simulink library "AEMS_Standard_Library"  (R2016b)
(part 13 of 39)

      | bit_ext_b7 = find_system(lib_path,'LookUnderMasks','all','FollowLinks','on','Name','DEM_LIB_BIT_EXTRACT7');
      | bit_ext_b8 = find_system(lib_path,'LookUnderMasks','all','FollowLinks','on','Name','DEM_LIB_BIT_EXTRACT8');
      | bit_ext_b0 = find_system(lib_path,'LookUnderMasks','all','FollowLinks','on','Name','DEM_LIB_BIT_EXTRACT0');
      | 
      | switch LibType
      |     case '_DGN'
      |         if ismember(get_param(bit_ext_b1,'MaskType'),{'AEMS_DEM_LIB_BIT_EXTRACT'})
      |         else
      |             replace_block(lib_path,'FollowLinks','on','Name','DEM_LIB_BIT_EXTRACT1','library/SUB/DEM_LIB_BIT_EXTRACT','noprompt');
      |             replace_block(lib_path,'FollowLinks','on','Name','DEM_LIB_BIT_EXTRACT2','library/SUB/DEM_LIB_BIT_EXTRACT','noprompt');
      |             replace_block(lib_path,'FollowLinks','on','Name','DEM_LIB_BIT_EXTRACT3','library/SUB/DEM_LIB_BIT_EXTRACT','noprompt');
      |             replace_block(lib_path,'FollowLinks','on','Name','DEM_LIB_BIT_EXTRACT4','library/SUB/DEM_LIB_BIT_EXTRACT','noprompt');
      |             replace_block(lib_path,'FollowLinks','on','Name','DEM_LIB_BIT_EXTRACT5','library/SUB/DEM_LIB_BIT_EXTRACT','noprompt');
      |             replace_block(lib_path,'FollowLinks','on','Name','DEM_LIB_BIT_EXTRACT6','library/SUB/DEM_LIB_BIT_EXTRACT','noprompt');
      |             replace_block(lib_path,'FollowLinks','on','Name','DEM_LIB_BIT_EXTRACT7','library/SUB/DEM_LIB_BIT_EXTRACT','noprompt');
      |             replace_block(lib_path,'FollowLinks','on','Name','DEM_LIB_BIT_EXTRACT8','library/SUB/DEM_LIB_BIT_EXTRACT','noprompt');
      |             replace_block(lib_path,'FollowLinks','on','Name','DEM_LIB_BIT_EXTRACT0','library/SUB/DEM_LIB_BIT_EXTRACT','noprompt');
      |         end
      |         set_param([bit_ext_b1{:}],'extract_bit','132');
      |         set_param([bit_ext_b2{:}],'extract_bit','132');
      |         set_param([bit_ext_b3{:}],'extract_bit','132');
      |         set_param([bit_ext_b4{:}],'extract_bit','132');
      |         set_param([bit_ext_b5{:}],'extract_bit','132');
      |         set_param([bit_ext_b6{:}],'extract_bit','132');
      |         set_param([bit_ext_b7{:}],'extract_bit','132');
      |         set_param([bit_ext_b8{:}],'extract_bit','132');
      |         set_param([bit_ext_b0{:}],'extract_bit','132');
      |     case '_FS(Hold at Key On)'
      |         if ismember(get_param(bit_ext_b1,'MaskType'),{'AEMS_DEM_LIB_BIT_EXTRACT'})
      |         else
      |             replace_block(lib_path,'FollowLinks','on','Name','DEM_LIB_BIT_EXTRACT1','library/SUB/DEM_LIB_BIT_EXTRACT','noprompt');
      |             replace_block(lib_path,'FollowLinks','on','Name','DEM_LIB_BIT_EXTRACT2','library/SUB/DEM_LIB_BIT_EXTRACT','noprompt');
      |             replace_block(lib_path,'FollowLinks','on','Name','DEM_LIB_BIT_EXTRACT3','library/SUB/DEM_LIB_BIT_EXTRACT','noprompt');
      |             replace_block(lib_path,'FollowLinks','on','Name','DEM_LIB_BIT_EXTRACT4','library/SUB/DEM_LIB_BIT_EXTRACT','noprompt');
      |             replace_block(lib_path,'FollowLinks','on','Name','DEM_LIB_BIT_EXTRACT5','library/SUB/DEM_LIB_BIT_EXTRACT','noprompt');
      |             replace_block(lib_path,'FollowLinks','on','Name','DEM_LIB_BIT_EXTRACT6','library/SUB/DEM_LIB_BIT_EXTRACT','noprompt');
      |             replace_block(lib_path,'FollowLinks','on','Name','DEM_LIB_BIT_EXTRACT7','library/SUB/DEM_LIB_BIT_EXTRACT','noprompt');
      |             replace_block(lib_path,'FollowLinks','on','Name','DEM_LIB_BIT_EXTRACT8','library/SUB/DEM_LIB_BIT_EXTRACT','noprompt');
      |             replace_block(lib_path,'FollowLinks','on','Name','DEM_LIB_BIT_EXTRACT0','library/SUB/DEM_LIB_BIT_EXTRACT','noprompt');
      |         end
      |         set_param([bit_ext_b1{:}],'extract_bit','1');
      |         set_param([bit_ext_b2{:}],'extract_bit','1');
      |         set_param([bit_ext_b3{:}],'extract_bit','1');
      |         set_param([bit_ext_b4{:}],'extract_bit','1');
      |         set_param([bit_ext_b5{:}],'extract_bit','1');
      |         set_param([bit_ext_b6{:}],'extract_bit','1');
      |         set_param([bit_ext_b7{:}],'extract_bit','1');
      |         set_param([bit_ext_b8{:}],'extract_bit','1');
      |         set_param([bit_ext_b0{:}],'extract_bit','1');
      |     case '_FS(Reset at Key On)'
      |         if ismember(get_param(bit_ext_b1,'MaskType'),{'AEMS_DEM_LIB_BIT_EXTRACT_FS_RESET'})
      |         else
      |             replace_block(lib_path,'FollowLinks','on','Name','DEM_LIB_BIT_EXTRACT1','library/SUB/DEM_LIB_BIT_EXTRACT_FS_RESET','noprompt');
      |             replace_block(lib_path,'FollowLinks','on','Name','DEM_LIB_BIT_EXTRACT2','library/SUB/DEM_LIB_BIT_EXTRACT_FS_RESET','noprompt');
      |             replace_block(lib_path,'FollowLinks','on','Name','DEM_LIB_BIT_EXTRACT3','library/SUB/DEM_LIB_BIT_EXTRACT_FS_RESET','noprompt');
      |             replace_block(lib_path,'FollowLinks','on','Name','DEM_LIB_BIT_EXTRACT4','library/SUB/DEM_LIB_BIT_EXTRACT_FS_RESET','noprompt');
      |             replace_block(lib_path,'FollowLinks','on','Name','DEM_LIB_BIT_EXTRACT5','library/SUB/DEM_LIB_BIT_EXTRACT_FS_RESET','noprompt');
      |             replace_block(lib_path,'FollowLinks','on','Name','DEM_LIB_BIT_EXTRACT6','library/SUB/DEM_LIB_BIT_EXTRACT_FS_RESET','noprompt');
      |             replace_block(lib_path,'FollowLinks','on','Name','DEM_LIB_BIT_EXTRACT7','library/SUB/DEM_LIB_BIT_EXTRACT_FS_RESET','noprompt');
      |             replace_block(lib_path,'FollowLinks','on','Name','DEM_LIB_BIT_EXTRACT8','library/SUB/DEM_LIB_BIT_EXTRACT_FS_RESET','noprompt');
      |             replace_block(lib_path,'FollowLinks','on','Name','DEM_LIB_BIT_EXTRACT0','library/SUB/DEM_LIB_BIT_EXTRACT_FS_RESET','noprompt');
      |         end
      |         set_param([bit_ext_b1{:}],'extract_bit1','1');
      |         set_param([bit_ext_b1{:}],'extract_bit2','64');
      |         set_param([bit_ext_b2{:}],'extract_bit1','1');
      |         set_param([bit_ext_b2{:}],'extract_bit2','64');
      |         set_param([bit_ext_b3{:}],'extract_bit1','1');
      |         set_param([bit_ext_b3{:}],'extract_bit2','64');
      |         set_param([bit_ext_b4{:}],'extract_bit1','1');
      |         set_param([bit_ext_b4{:}],'extract_bit2','64');
      |         set_param([bit_ext_b5{:}],'extract_bit1','1');
      |         set_param([bit_ext_b5{:}],'extract_bit2','64');
      |         set_param([bit_ext_b6{:}],'extract_bit1','1');
      |         set_param([bit_ext_b6{:}],'extract_bit2','64');
      |         set_param([bit_ext_b7{:}],'extract_bit1','1');
      |         set_param([bit_ext_b7{:}],'extract_bit2','64');
      |         set_param([bit_ext_b8{:}],'extract_bit1','1');
      |         set_param([bit_ext_b8{:}],'extract_bit2','64');
      |         set_param([bit_ext_b0{:}],'extract_bit1','1');
      |         set_param([bit_ext_b0{:}],'extract_bit2','64');
      |     case '_NBC'
      |         if ismember(get_param(bit_ext_b1,'MaskType'),{'AEMS_DEM_LIB_BIT_EXTRACT'})
      |         else
      |             replace_block(lib_path,'FollowLinks','on','Name','DEM_LIB_BIT_EXTRACT1','library/SUB/DEM_LIB_BIT_EXTRACT','noprompt');
      |             replace_block(lib_path,'FollowLinks','on','Name','DEM_LIB_BIT_EXTRACT2','library/SUB/DEM_LIB_BIT_EXTRACT','noprompt');
      |             replace_block(lib_path,'FollowLinks','on','Name','DEM_LIB_BIT_EXTRACT3','library/SUB/DEM_LIB_BIT_EXTRACT','noprompt');
      |             replace_block(lib_path,'FollowLinks','on','Name','DEM_LIB_BIT_EXTRACT4','library/SUB/DEM_LIB_BIT_EXTRACT','noprompt');
      |             replace_block(lib_path,'FollowLinks','on','Name','DEM_LIB_BIT_EXTRACT5','library/SUB/DEM_LIB_BIT_EXTRACT','noprompt');
      |             replace_block(lib_path,'FollowLinks','on','Name','DEM_LIB_BIT_EXTRACT6','library/SUB/DEM_LIB_BIT_EXTRACT','noprompt');
      |             replace_block(lib_path,'FollowLinks','on','Name','DEM_LIB_BIT_EXTRACT7','library/SUB/DEM_LIB_BIT_EXTRACT','noprompt');
      |             replace_block(lib_path,'FollowLinks','on','Name','DEM_LIB_BIT_EXTRACT8','library/SUB/DEM_LIB_BIT_EXTRACT','noprompt');
      |             replace_block(lib_path,'FollowLinks','on','Name','DEM_LIB_BIT_EXTRACT0','library/SUB/DEM_LIB_BIT_EXTRACT','noprompt');
      |         end
      |         set_param([bit_ext_b1{:}],'extract_bit','2');
      |         set_param([bit_ext_b2{:}],'extract_bit','2');
      |         set_param([bit_ext_b3{:}],'extract_bit','2');
      |         set_param([bit_ext_b4{:}],'extract_bit','2');
      |         set_param([bit_ext_b5{:}],'extract_bit','2');
      |         set_param([bit_ext_b6{:}],'extract_bit','2');
      |         set_param([bit_ext_b7{:}],'extract_bit','2');
      |         set_param([bit_ext_b8{:}],'extract_bit','2');
      |         set_param([bit_ext_b0{:}],'extract_bit','2');
      |     case '_NGBU'
      |         if ismember(get_param(bit_ext_b1,'MaskType'),{'AEMS_DEM_LIB_BIT_EXTRACT'})
      |         else
      |             replace_block(lib_path,'FollowLinks','on','Name','DEM_LIB_BIT_EXTRACT1','library/SUB/DEM_LIB_BIT_EXTRACT','noprompt');
      |             replace_block(lib_path,'FollowLinks','on','Name','DEM_LIB_BIT_EXTRACT2','library/SUB/DEM_LIB_BIT_EXTRACT','noprompt');
      |             replace_block(lib_path,'FollowLinks','on','Name','DEM_LIB_BIT_EXTRACT3','library/SUB/DEM_LIB_BIT_EXTRACT','noprompt');
      |             replace_block(lib_path,'FollowLinks','on','Name','DEM_LIB_BIT_EXTRACT4','library/SUB/DEM_LIB_BIT_EXTRACT','noprompt');
      |             replace_block(lib_path,'FollowLinks','on','Name','DEM_LIB_BIT_EXTRACT5','library/SUB/DEM_LIB_BIT_EXTRACT','noprompt');
      |             replace_block(lib_path,'FollowLinks','on','Name','DEM_LIB_BIT_EXTRACT6','library/SUB/DEM_LIB_BIT_EXTRACT','noprompt');
      |             replace_block(lib_path,'FollowLinks','on','Name','DEM_LIB_BIT_EXTRACT7','library/SUB/DEM_LIB_BIT_EXTRACT','noprompt');
      |             replace_block(lib_path,'FollowLinks','on','Name','DEM_LIB_BIT_EXTRACT8','library/SUB/DEM_LIB_BIT_EXTRACT','noprompt');
      |             replace_block(lib_path,'FollowLinks','on','Name','DEM_LIB_BIT_EXTRACT0','library/SUB/DEM_LIB_BIT_EXTRACT','noprompt');
      |         end
      |         set_param([bit_ext_b1{:}],'extract_bit','4');
      |         set_param([bit_ext_b2{:}],'extract_bit','4');
      |         set_param([bit_ext_b3{:}],'extract_bit','4');
      |         set_param([bit_ext_b4{:}],'extract_bit','4');
      |         set_param([bit_ext_b5{:}],'extract_bit','4');
      |         set_param([bit_ext_b6{:}],'extract_bit','4');
      |         set_param([bit_ext_b7{:}],'extract_bit','4');
      |         set_param([bit_ext_b8{:}],'extract_bit','4');
      |         set_param([bit_ext_b0{:}],'extract_bit','4');
      |     case '_M7NGBU'
      |         if ismember(get_param(bit_ext_b1,'MaskType'),{'AEMS_DEM_LIB_BIT_EXTRACT'})
      |         else
      |             replace_block(lib_path,'FollowLinks','on','Name','DEM_LIB_BIT_EXTRACT1','library/SUB/DEM_LIB_BIT_EXTRACT','noprompt');
      |             replace_block(lib_path,'FollowLinks','on','Name','DEM_LIB_BIT_EXTRACT2','library/SUB/DEM_LIB_BIT_EXTRACT','noprompt');
      |             replace_block(lib_path,'FollowLinks','on','Name','DEM_LIB_BIT_EXTRACT3','library/SUB/DEM_LIB_BIT_EXTRACT','noprompt');
      |             replace_block(lib_path,'FollowLinks','on','Name','DEM_LIB_BIT_EXTRACT4','library/SUB/DEM_LIB_BIT_EXTRACT','noprompt');
      |             replace_block(lib_path,'FollowLinks','on','Name','DEM_LIB_BIT_EXTRACT5','library/SUB/DEM_LIB_BIT_EXTRACT','noprompt');
      |             replace_block(lib_path,'FollowLinks','on','Name','DEM_LIB_BIT_EXTRACT6','library/SUB/DEM_LIB_BIT_EXTRACT','noprompt');
      |             replace_block(lib_path,'FollowLinks','on','Name','DEM_LIB_BIT_EXTRACT7','library/SUB/DEM_LIB_BIT_EXTRACT','noprompt');
      |             replace_block(lib_path,'FollowLinks','on','Name','DEM_LIB_BIT_EXTRACT8','library/SUB/DEM_LIB_BIT_EXTRACT','noprompt');
      |             replace_block(lib_path,'FollowLinks','on','Name','DEM_LIB_BIT_EXTRACT0','library/SUB/DEM_LIB_BIT_EXTRACT','noprompt');
      |         end
      |         set_param([bit_ext_b1{:}],'extract_bit','4');
      |         set_param([bit_ext_b2{:}],'extract_bit','4');
      |         set_param([bit_ext_b3{:}],'extract_bit','4');
      |         set_param([bit_ext_b4{:}],'extract_bit','4');
      |         set_param([bit_ext_b5{:}],'extract_bit','4');
      |         set_param([bit_ext_b6{:}],'extract_bit','4');
      |         set_param([bit_ext_b7{:}],'extract_bit','4');
      |         set_param([bit_ext_b8{:}],'extract_bit','4');
      |         set_param([bit_ext_b0{:}],'extract_bit','4');
      |     case '_NGREM'
      |         if ismember(get_param(bit_ext_b1,'MaskType'),{'AEMS_DEM_LIB_BIT_EXTRACT'})
      |         else
      |             replace_block(lib_path,'FollowLinks','on','Name','DEM_LIB_BIT_EXTRACT1','library/SUB/DEM_LIB_BIT_EXTRACT','noprompt');
      |             replace_block(lib_path,'FollowLinks','on','Name','DEM_LIB_BIT_EXTRACT2','library/SUB/DEM_LIB_BIT_EXTRACT','noprompt');
      |             replace_block(lib_path,'FollowLinks','on','Name','DEM_LIB_BIT_EXTRACT3','library/SUB/DEM_LIB_BIT_EXTRACT','noprompt');
      |             replace_block(lib_path,'FollowLinks','on','Name','DEM_LIB_BIT_EXTRACT4','library/SUB/DEM_LIB_BIT_EXTRACT','noprompt');
      |             replace_block(lib_path,'FollowLinks','on','Name','DEM_LIB_BIT_EXTRACT5','library/SUB/DEM_LIB_BIT_EXTRACT','noprompt');
      |             replace_block(lib_path,'FollowLinks','on','Name','DEM_LIB_BIT_EXTRACT6','library/SUB/DEM_LIB_BIT_EXTRACT','noprompt');
      |             replace_block(lib_path,'FollowLinks','on','Name','DEM_LIB_BIT_EXTRACT7','library/SUB/DEM_LIB_BIT_EXTRACT','noprompt');
      |             replace_block(lib_path,'FollowLinks','on','Name','DEM_LIB_BIT_EXTRACT8','library/SUB/DEM_LIB_BIT_EXTRACT','noprompt');
      |             replace_block(lib_path,'FollowLinks','on','Name','DEM_LIB_BIT_EXTRACT0','library/SUB/DEM_LIB_BIT_EXTRACT','noprompt');
      |         end
      |         set_param([bit_ext_b1{:}],'extract_bit','8');
      |         set_param([bit_ext_b2{:}],'extract_bit','8');
      |         set_param([bit_ext_b3{:}],'extract_bit','8');
      |         set_param([bit_ext_b4{:}],'extract_bit','8');
      |         set_param([bit_ext_b5{:}],'extract_bit','8');
      |         set_param([bit_ext_b6{:}],'extract_bit','8');
      |         set_param([bit_ext_b7{:}],'extract_bit','8');
      |         set_param([bit_ext_b8{:}],'extract_bit','8');
      |         set_param([bit_ext_b0{:}],'extract_bit','8');
      |     case '_NGMEM'
      |         if ismember(get_param(bit_ext_b1,'MaskType'),{'AEMS_DEM_LIB_BIT_EXTRACT'})
      |         else
      |             replace_block(lib_path,'FollowLinks','on','Name','DEM_LIB_BIT_EXTRACT1','library/SUB/DEM_LIB_BIT_EXTRACT','noprompt');
      |             replace_block(lib_path,'FollowLinks','on','Name','DEM_LIB_BIT_EXTRACT2','library/SUB/DEM_LIB_BIT_EXTRACT','noprompt');
      |             replace_block(lib_path,'FollowLinks','on','Name','DEM_LIB_BIT_EXTRACT3','library/SUB/DEM_LIB_BIT_EXTRACT','noprompt');
      |             replace_block(lib_path,'FollowLinks','on','Name','DEM_LIB_BIT_EXTRACT4','library/SUB/DEM_LIB_BIT_EXTRACT','noprompt');
      |             replace_block(lib_path,'FollowLinks','on','Name','DEM_LIB_BIT_EXTRACT5','library/SUB/DEM_LIB_BIT_EXTRACT','noprompt');
      |             replace_block(lib_path,'FollowLinks','on','Name','DEM_LIB_BIT_EXTRACT6','library/SUB/DEM_LIB_BIT_EXTRACT','noprompt');
      |             replace_block(lib_path,'FollowLinks','on','Name','DEM_LIB_BIT_EXTRACT7','library/SUB/DEM_LIB_BIT_EXTRACT','noprompt');
      |             replace_block(lib_path,'FollowLinks','on','Name','DEM_LIB_BIT_EXTRACT8','library/SUB/DEM_LIB_BIT_EXTRACT','noprompt');
      |             replace_block(lib_path,'FollowLinks','on','Name','DEM_LIB_BIT_EXTRACT0','library/SUB/DEM_LIB_BIT_EXTRACT','noprompt');
      |         end
      |         set_param([bit_ext_b1{:}],'extract_bit','32');
      |         set_param([bit_ext_b2{:}],'extract_bit','32');
      |         set_param([bit_ext_b3{:}],'extract_bit','32');
      |         set_param([bit_ext_b4{:}],'extract_bit','32');
      |         set_param([bit_ext_b5{:}],'extract_bit','32');
      |         set_param([bit_ext_b6{:}],'extract_bit','32');
      |         set_param([bit_ext_b7{:}],'extract_bit','32');
      |         set_param([bit_ext_b8{:}],'extract_bit','32');
      |         set_param([bit_ext_b0{:}],'extract_bit','32');
      |     case '_MIL'
      |         if ismember(get_param(bit_ext_b1,'MaskType'),{'AEMS_DEM_LIB_BIT_EXTRACT'})
      |         else
      |             replace_block(lib_path,'FollowLinks','on','Name','DEM_LIB_BIT_EXTRACT1','library/SUB/DEM_LIB_BIT_EXTRACT','noprompt');
      |             replace_block(lib_path,'FollowLinks','on','Name','DEM_LIB_BIT_EXTRACT2','library/SUB/DEM_LIB_BIT_EXTRACT','noprompt');
      |             replace_block(lib_path,'FollowLinks','on','Name','DEM_LIB_BIT_EXTRACT3','library/SUB/DEM_LIB_BIT_EXTRACT','noprompt');
      |             replace_block(lib_path,'FollowLinks','on','Name','DEM_LIB_BIT_EXTRACT4','library/SUB/DEM_LIB_BIT_EXTRACT','noprompt');
      |             replace_block(lib_path,'FollowLinks','on','Name','DEM_LIB_BIT_EXTRACT5','library/SUB/DEM_LIB_BIT_EXTRACT','noprompt');
      |             replace_block(lib_path,'FollowLinks','on','Name','DEM_LIB_BIT_EXTRACT6','library/SUB/DEM_LIB_BIT_EXTRACT','noprompt');
      |             replace_block(lib_path,'FollowLinks','on','Name','DEM_LIB_BIT_EXTRACT7','library/SUB/DEM_LIB_BIT_EXTRACT','noprompt');
      |             replace_block(lib_path,'FollowLinks','on','Name','DEM_LIB_BIT_EXTRACT8','library/SUB/DEM_LIB_BIT_EXTRACT','noprompt');
      |             replace_block(lib_path,'FollowLinks','on','Name','DEM_LIB_BIT_EXTRACT0','library/SUB/DEM_LIB_BIT_EXTRACT','noprompt');
      |         end
      |         set_param([bit_ext_b1{:}],'extract_bit','128');
      |         set_param([bit_ext_b2{:}],'extract_bit','128');
      |         set_param([bit_ext_b3{:}],'extract_bit','128');
      |         set_param([bit_ext_b4{:}],'extract_bit','128');
      |         set_param([bit_ext_b5{:}],'extract_bit','128');
      |         set_param([bit_ext_b6{:}],'extract_bit','128');
      |         set_param([bit_ext_b7{:}],'extract_bit','128');
      |         set_param([bit_ext_b8{:}],'extract_bit','128');
      |         set_param([bit_ext_b0{:}],'extract_bit','128');
      |     case '_FMILON'
      |         if ismember(get_param(bit_ext_b1,'MaskType'),{'AEMS_DEM_LIB_BIT_EXTRACT'})
      |         else
      |             replace_block(lib_path,'FollowLinks','on','Name','DEM_LIB_BIT_EXTRACT1','library/SUB/DEM_LIB_BIT_EXTRACT','noprompt');
      |             replace_block(lib_path,'FollowLinks','on','Name','DEM_LIB_BIT_EXTRACT2','library/SUB/DEM_LIB_BIT_EXTRACT','noprompt');
      |             replace_block(lib_path,'FollowLinks','on','Name','DEM_LIB_BIT_EXTRACT3','library/SUB/DEM_LIB_BIT_EXTRACT','noprompt');
      |             replace_block(lib_path,'FollowLinks','on','Name','DEM_LIB_BIT_EXTRACT4','library/SUB/DEM_LIB_BIT_EXTRACT','noprompt');
      |             replace_block(lib_path,'FollowLinks','on','Name','DEM_LIB_BIT_EXTRACT5','library/SUB/DEM_LIB_BIT_EXTRACT','noprompt');
      |             replace_block(lib_path,'FollowLinks','on','Name','DEM_LIB_BIT_EXTRACT6','library/SUB/DEM_LIB_BIT_EXTRACT','noprompt');
      |             replace_block(lib_path,'FollowLinks','on','Name','DEM_LIB_BIT_EXTRACT7','library/SUB/DEM_LIB_BIT_EXTRACT','noprompt');
      |             replace_block(lib_path,'FollowLinks','on','Name','DEM_LIB_BIT_EXTRACT8','library/SUB/DEM_LIB_BIT_EXTRACT','noprompt');
      |             replace_block(lib_path,'FollowLinks','on','Name','DEM_LIB_BIT_EXTRACT0','library/SUB/DEM_LIB_BIT_EXTRACT','noprompt');
      |         end
      |         set_param([bit_ext_b1{:}],'extract_bit','128');
      |         set_param([bit_ext_b2{:}],'extract_bit','128');
      |         set_param([bit_ext_b3{:}],'extract_bit','128');
      |         set_param([bit_ext_b4{:}],'extract_bit','128');
      |         set_param([bit_ext_b5{:}],'extract_bit','128');
      |         set_param([bit_ext_b6{:}],'extract_bit','128');
      |         set_param([bit_ext_b7{:}],'extract_bit','128');
      |         set_param([bit_ext_b8{:}],'extract_bit','128');
      |         set_param([bit_ext_b0{:}],'extract_bit','128');
      |     case '_FDGNOK'
      |         if ismember(get_param(bit_ext_b1,'MaskType'),{'AEMS_DEM_LIB_BIT_EXTRACT_FDGNOK'})
      |         else
      |             replace_block(lib_path,'FollowLinks','on','Name','DEM_LIB_BIT_EXTRACT1','library/SUB/DEM_LIB_BIT_EXTRACT_FDGNOK','noprompt');
      |             replace_block(lib_path,'FollowLinks','on','Name','DEM_LIB_BIT_EXTRACT2','library/SUB/DEM_LIB_BIT_EXTRACT_FDGNOK','noprompt');
      |             replace_block(lib_path,'FollowLinks','on','Name','DEM_LIB_BIT_EXTRACT3','library/SUB/DEM_LIB_BIT_EXTRACT_FDGNOK','noprompt');
      |             replace_block(lib_path,'FollowLinks','on','Name','DEM_LIB_BIT_EXTRACT4','library/SUB/DEM_LIB_BIT_EXTRACT_FDGNOK','noprompt');
      |             replace_block(lib_path,'FollowLinks','on','Name','DEM_LIB_BIT_EXTRACT5','library/SUB/DEM_LIB_BIT_EXTRACT_FDGNOK','noprompt');
      |             replace_block(lib_path,'FollowLinks','on','Name','DEM_LIB_BIT_EXTRACT6','library/SUB/DEM_LIB_BIT_EXTRACT_FDGNOK','noprompt');
      |             replace_block(lib_path,'FollowLinks','on','Name','DEM_LIB_BIT_EXTRACT7','library/SUB/DEM_LIB_BIT_EXTRACT_FDGNOK','noprompt');
      |             replace_block(lib_path,'FollowLinks','on','Name','DEM_LIB_BIT_EXTRACT8','library/SUB/DEM_LIB_BIT_EXTRACT_FDGNOK','noprompt');
      |             replace_block(lib_path,'FollowLinks','on','Name','DEM_LIB_BIT_EXTRACT0','library/SUB/DEM_LIB_BIT_EXTRACT_FDGNOK','noprompt');
      |         end
      |         set_param([bit_ext_b1{:}],'extract_bit1','2');
      |         set_param([bit_ext_b1{:}],'extract_bit2','64');
      |         set_param([bit_ext_b2{:}],'extract_bit1','2');
      |         set_param([bit_ext_b2{:}],'extract_bit2','64');
      |         set_param([bit_ext_b3{:}],'extract_bit1','2');
      |         set_param([bit_ext_b3{:}],'extract_bit2','64');
      |         set_param([bit_ext_b4{:}],'extract_bit1','2');
      |         set_param([bit_ext_b4{:}],'extract_bit2','64');
      |         set_param([bit_ext_b5{:}],'extract_bit1','2');
      |         set_param([bit_ext_b5{:}],'extract_bit2','64');
      |         set_param([bit_ext_b6{:}],'extract_bit1','2');
      |         set_param([bit_ext_b6{:}],'extract_bit2','64');
      |         set_param([bit_ext_b7{:}],'extract_bit1','2');
      |         set_param([bit_ext_b7{:}],'extract_bit2','64');
      |         set_param([bit_ext_b8{:}],'extract_bit1','2');
      |         set_param([bit_ext_b8{:}],'extract_bit2','64');
      |         set_param([bit_ext_b0{:}],'extract_bit1','2');
      |         set_param([bit_ext_b0{:}],'extract_bit2','64');
      |     case '_MEM'
      |         if ismember(get_param(bit_ext_b1,'MaskType'),{'AEMS_DEM_LIB_BIT_EXTRACT'})
      |         else
      |             replace_block(lib_path,'FollowLinks','on','Name','DEM_LIB_BIT_EXTRACT1','library/SUB/DEM_LIB_BIT_EXTRACT','noprompt');
      |             replace_block(lib_path,'FollowLinks','on','Name','DEM_LIB_BIT_EXTRACT2','library/SUB/DEM_LIB_BIT_EXTRACT','noprompt');
      |             replace_block(lib_path,'FollowLinks','on','Name','DEM_LIB_BIT_EXTRACT3','library/SUB/DEM_LIB_BIT_EXTRACT','noprompt');
      |             replace_block(lib_path,'FollowLinks','on','Name','DEM_LIB_BIT_EXTRACT4','library/SUB/DEM_LIB_BIT_EXTRACT','noprompt');
      |             replace_block(lib_path,'FollowLinks','on','Name','DEM_LIB_BIT_EXTRACT5','library/SUB/DEM_LIB_BIT_EXTRACT','noprompt');
      |             replace_block(lib_path,'FollowLinks','on','Name','DEM_LIB_BIT_EXTRACT6','library/SUB/DEM_LIB_BIT_EXTRACT','noprompt');
      |             replace_block(lib_path,'FollowLinks','on','Name','DEM_LIB_BIT_EXTRACT7','library/SUB/DEM_LIB_BIT_EXTRACT','noprompt');
      |             replace_block(lib_path,'FollowLinks','on','Name','DEM_LIB_BIT_EXTRACT8','library/SUB/DEM_LIB_BIT_EXTRACT','noprompt');
      |             replace_block(lib_path,'FollowLinks','on','Name','DEM_LIB_BIT_EXTRACT0','library/SUB/DEM_LIB_BIT_EXTRACT','noprompt');
      |         end
      |         set_param([bit_ext_b1{:}],'extract_bit','32');
      |         set_param([bit_ext_b2{:}],'extract_bit','32');
      |         set_param([bit_ext_b3{:}],'extract_bit','32');
      |         set_param([bit_ext_b4{:}],'extract_bit','32');
      |         set_param([bit_ext_b5{:}],'extract_bit','32');
      |         set_param([bit_ext_b6{:}],'extract_bit','32');
      |         set_param([bit_ext_b7{:}],'extract_bit','32');
      |         set_param([bit_ext_b8{:}],'extract_bit','32');
      |         set_param([bit_ext_b0{:}],'extract_bit','32');
      |     case '_FLGMEM'
      |         if ismember(get_param(bit_ext_b1,'MaskType'),{'AEMS_DEM_LIB_BIT_EXTRACT'})
      |         else
      |             replace_block(lib_path,'FollowLinks','on','Name','DEM_LIB_BIT_EXTRACT1','library/SUB/DEM_LIB_BIT_EXTRACT','noprompt');
      |             replace_block(lib_path,'FollowLinks','on','Name','DEM_LIB_BIT_EXTRACT2','library/SUB/DEM_LIB_BIT_EXTRACT','noprompt');
      |             replace_block(lib_path,'FollowLinks','on','Name','DEM_LIB_BIT_EXTRACT3','library/SUB/DEM_LIB_BIT_EXTRACT','noprompt');
      |             replace_block(lib_path,'FollowLinks','on','Name','DEM_LIB_BIT_EXTRACT4','library/SUB/DEM_LIB_BIT_EXTRACT','noprompt');
      |             replace_block(lib_path,'FollowLinks','on','Name','DEM_LIB_BIT_EXTRACT5','library/SUB/DEM_LIB_BIT_EXTRACT','noprompt');
      |             replace_block(lib_path,'FollowLinks','on','Name','DEM_LIB_BIT_EXTRACT6','library/SUB/DEM_LIB_BIT_EXTRACT','noprompt');
      |             replace_block(lib_path,'FollowLinks','on','Name','DEM_LIB_BIT_EXTRACT7','library/SUB/DEM_LIB_BIT_EXTRACT','noprompt');
      |             replace_block(lib_path,'FollowLinks','on','Name','DEM_LIB_BIT_EXTRACT8','library/SUB/DEM_LIB_BIT_EXTRACT','noprompt');
      |             replace_block(lib_path,'FollowLinks','on','Name','DEM_LIB_BIT_EXTRACT0','library/SUB/DEM_LIB_BIT_EXTRACT','noprompt');
      |         end
      |         set_param([bit_ext_b1{:}],'extract_bit','32');
      |         set_param([bit_ext_b2{:}],'extract_bit','32');
      |         set_param([bit_ext_b3{:}],'extract_bit','32');
      |         set_param([bit_ext_b4{:}],'extract_bit','32');
      |         set_param([bit_ext_b5{:}],'extract_bit','32');
      |         set_param([bit_ext_b6{:}],'extract_bit','32');
      |         set_param([bit_ext_b7{:}],'extract_bit','32');
      |         set_param([bit_ext_b8{:}],'extract_bit','32');
      |         set_param([bit_ext_b0{:}],'extract_bit','32');
      | end
      settings: AttributesFormatString=%<MaskType>\nEventId : = %<EventId>\nDEM Library type : = %<LibType>\nFunction Mode : = %<FunctionMode>
      mask TypeOptions LibType: _DGN | _FS(Hold at Key On) | _FS(Reset at Key On) | _NBC | _NGBU | _M7NGBU | _NGREM | _NGMEM | _MIL | _FMILON | _FDGNOK | _MEM | _FLGMEM
      mask TypeOptions FunctionMode: Dysfunctional | From Data Store memory
      mask Display:
      | dgn_mask = ['Event ID: ' char(EventId) '\n Library type: ' char(LibType)];
      | 
      | disp(dgn_mask);
      | plot([5,5,5])
      | plot([6,6,6])
  AEMS_DEM_LIB_BIT_EXTRACT : Subsystem  Tag=[LIB]  mask(AEMS_DEM_LIB_BIT_EXTRACT){extract_bit=4}
      mask init:
      | check_bit = get_param(gcb,'extract_bit');
      | set_param([gcb '/bit_check'],'Value',check_bit);
      settings: AttributesFormatString=%<MaskType>\nextract_bit = %<extract_bit>
      mask Display:
      | % disp(sprintf('Bit %s', char(name)))
      | mask_disp = ['BIT EXTRACT \n [ ' dec2bin(extract_bit,8) ' ]'];
      | disp(mask_disp);
      | plot([5,5,5])
      | plot([6,6,6])
  AEMS_DEM_LIB_BIT_EXTRACT_FDGNOK : Subsystem  Tag=[LIB]  mask(AEMS_DEM_LIB_BIT_EXTRACT_FDGNOK){extract_bit1=2, extract_bit2=64}
      mask help: DEM_LIB_BIT_EXTRACT for [_FDGNOK]
      mask init:
      | check_bit1 = get_param(gcb,'extract_bit1');
      | check_bit2 = get_param(gcb,'extract_bit2');
      | set_param([gcb '/bit_check1'],'Value',check_bit1);
      | set_param([gcb '/bit_check2'],'Value',check_bit2);
      settings: AttributesFormatString=%<MaskType>\nextract_bit1 = %<extract_bit1>\nextract_bit2 = %<extract_bit2>
      mask Display:
      | mask_disp = ['BIT EXTRACT FDGNOK\n[ ' dec2bin(extract_bit1,8) ' ]\n[ ' dec2bin(extract_bit2,8) ' ]'];
      | disp(mask_disp);
      | plot([5,5,5])
      | plot([6,6,6])
  AEMS_DEM_LIB_BIT_EXTRACT_FS_RESET : Subsystem  Tag=[LIB]  mask(AEMS_DEM_LIB_BIT_EXTRACT_FS_RESET){extract_bit1=1, extract_bit2=64}
      mask init:
      | check_bit1 = get_param(gcb,'extract_bit1');
      | check_bit2 = get_param(gcb,'extract_bit2');
      | set_param([gcb '/bit_check1'],'Value',check_bit1);
      | set_param([gcb '/bit_check2'],'Value',check_bit2);
      settings: AttributesFormatString=%<MaskType>\nextract_bit1 = %<extract_bit1>\nextract_bit2 = %<extract_bit2>
      mask Display:
      | mask_disp = ['BIT EXTRACT FS(Reset)\n[ ' dec2bin(extract_bit1,8) ' ]\n[ ' dec2bin(extract_bit2,8) ' ]'];
      | disp(mask_disp);
      | plot([5,5,5])
      | plot([6,6,6])
  AEMS_DEM_READDATAOFPID01 : Subsystem  Tag=[LIB]  mask(AEMS_DEM_READDATAOFPID01){}
      mask help:
      | This library calls AUTOSAR standard functions.
      | To know more details, please refer AUTOSAR DEM01167.
      settings: AttributesFormatString=%<MaskType>
      mask Display:
      | disp(['Dem_ReadDataOfPID01 \n \n \n \n \n']);
      | plot([5,5,5])
      | plot([6,6,6])
      | 
      | port_label('output',1,'vPID01')
  AEMS_DEM_REPIUMPRDENLOCK : Subsystem  Tag=[LIB]  mask(AEMS_DEM_REPIUMPRDENLOCK){}
      mask help:
      | This library calls AUTOSAR standard functions.
      | To know more details, please refer AUTOSAR DEM00314.
      settings: AttributesFormatString=%<MaskType>
      mask Display:
      | disp(['Dem_RepIUMPRDenLock \n \n \n \n \n']);
      | plot([5,5,5])
      | plot([6,6,6])
      | port_label('input',1,'RatioId')
  AEMS_DEM_REPIUMPRDENRELEASE : Subsystem  Tag=[LIB]  mask(AEMS_DEM_REPIUMPRDENRELEASE){}
      mask help:
      | This library calls AUTOSAR standard functions.
      | To know more details, please refer AUTOSAR DEM00315.
      settings: AttributesFormatString=%<MaskType>
      mask Display:
      | disp(['Dem_RepIUMPRDenRelease \n \n \n \n \n']);
      | plot([5,5,5])
      | plot([6,6,6])
      | port_label('input',1,'RatioId')
  AEMS_DEM_REPIUMPRFAULTDETECT : Subsystem  Tag=[LIB]  mask(AEMS_DEM_REPIUMPRFAULTDETECT){}
      mask help:
      | This library calls AUTOSAR standard functions.
      | To know more details, please refer AUTOSAR DEM00313.
      settings: AttributesFormatString=%<MaskType>
      mask Display:
      | disp(['Dem_RepIUMPRFaultDetect \n \n \n \n \n']);
      | plot([5,5,5])
      | plot([6,6,6])
      | port_label('input',1,'RatioId')
  AEMS_DEM_REP_IUMPR_1D : Subsystem  Tag=[LIB]  mask(AEMS_DEM_REP_IUMPR_1D){RatioId=Dem_RatioId_XXX}
      mask prompts: RatioId "RatioId :"
      mask init:
      | eval([char(RatioId), ' = 0;']);
      | 
      | ratioid_b1 = find_system(gcb,'LookUnderMasks','all','FollowLinks','on','Name','RatioId_block1');
      | 
      | % 3sets(FaultDetect/DenLock/DenRelease)
      | for n = 1:length(ratioid_b1)
      |     set_param([ratioid_b1{n}],'Value',char(RatioId));
      | end
      settings: AttributesFormatString=%<MaskType>\nRatioId : = %<RatioId>
      mask Display:
      | % dgn_mask = ['Diagnosis name: ' char(DiagName) '\n Ratio ID: ' char(RatioId) ];
      | dgn_mask = ['Ratio ID: ' char(RatioId) ];
      | disp(dgn_mask);
      | port_label('input',1,'denlock_status');
      | port_label('input',2,'faultdetect_trigger');
      | 
      | plot([5,5,5])
      | plot([6,6,6])
  AEMS_DEM_REP_IUMPR_2D : Subsystem  Tag=[LIB]  mask(AEMS_DEM_REP_IUMPR_2D){RatioId=Dem_RatioId_XXX}
      mask prompts: RatioId "RatioId :"
      mask init:
      | % eval([char(RatioId), '_1 = 0;']);
      | % eval([char(RatioId), '_2 = 0;']);
      | 
      | ratioid_b1 = find_system(gcb,'LookUnderMasks','all','FollowLinks','on','Name','RatioId_block1');
      | ratioid_b2 = find_system(gcb,'LookUnderMasks','all','FollowLinks','on','Name','RatioId_block2');
      | ratio_id = get_param(gcb,'RatioId');
      | % 3sets(FaultDetect/DenLock/DenRelease)
      | for n = 1:length(ratioid_b1)
      | %     set_param([ratioid_b1{n}],'Value',[char(RatioId) '_1']);
      | %     set_param([ratioid_b2{n}],'Value',[char(RatioId) '_2']);
      |         eval([char(ratio_id), '= 0;']);        
      |         set_param([ratioid_b1{n}],'Value',ratio_id);
      |         Splitname=regexp(ratio_id,'_','all');
      |         ratioId=insertBefore(ratio_id,Splitname(end),'2');
      |         eval([char(ratioId), '= 0;']);
      |         set_param([ratioid_b2{n}],'Value',ratioId);
      | end
      settings: AttributesFormatString=%<MaskType>\nRatioId : = %<RatioId>
      mask Display:
      | % dgn_mask = ['Diagnosis name: ' char(DiagName) '\n Ratio ID: ' char(RatioId) ];
      | dgn_mask = ['Ratio ID: ' char(RatioId) ];
      | 
      | disp(dgn_mask);
      | port_label('input',1,'denlock_status');
      | port_label('input',2,'faultdetect_trigger');
      | 
      | plot([5,5,5])
      | plot([6,6,6])
  AEMS_DEM_REP_IUMPR_8D : Subsystem  Tag=[LIB]  mask(AEMS_DEM_REP_IUMPR_8D){RatioId=Dem_RatioId_XXX}
      mask prompts: RatioId "RatioId :"
      mask init:
      | Lib_path=gcb;
      | ratioid_b1 = find_system(Lib_path,'LookUnderMasks','all','FollowLinks','on','Name','RatioId_block1');
      | ratioid_b2 = find_system(Lib_path,'LookUnderMasks','all','FollowLinks','on','Name','RatioId_block2');
      | ratioid_b3 = find_system(Lib_path,'LookUnderMasks','all','FollowLinks','on','Name','RatioId_block3');
      | ratioid_b4 = find_system(Lib_path,'LookUnderMasks','all','FollowLinks','on','Name','RatioId_block4');
      | ratioid_b5 = find_system(Lib_path,'LookUnderMasks','all','FollowLinks','on','Name','RatioId_block5');
      | ratioid_b6 = find_system(Lib_path,'LookUnderMasks','all','FollowLinks','on','Name','RatioId_block6');
      | ratioid_b7 = find_system(Lib_path,'LookUnderMasks','all','FollowLinks','on','Name','RatioId_block7');
      | ratioid_b8 = find_system(Lib_path,'LookUnderMasks','all','FollowLinks','on','Name','RatioId_block8');
      | ratio_id = get_param(Lib_path,'RatioId');
      | % 3sets(FaultDetect/DenLock/DenRelease)
      | for n = 1:length(ratioid_b1)
      |     eval([char(ratio_id), '= 0;']);
      |     set_param([ratioid_b1{n}],'Value',ratio_id);
      |     
      |     Splitname=regexp(ratio_id,'_','all');
      |     ratioId=insertBefore(ratio_id,Splitname(end),'2');
      |     eval([char(ratioId), '= 0;']);
      |     set_param([ratioid_b2{n}],'Value',ratioId);
      |     
      |     Splitname=regexp(ratio_id,'_','all');
      |     ratioId=insertBefore(ratio_id,Splitname(end),'3');
      |     eval([char(ratioId), '= 0;']);
      |     set_param([ratioid_b3{n}],'Value',ratioId);
      |     
      |     Splitname=regexp(ratio_id,'_','all');
      |     ratioId=insertBefore(ratio_id,Splitname(end),'4');
      |     eval([char(ratioId), '= 0;']);
      |     set_param([ratioid_b4{n}],'Value',ratioId);
      |     
      |     Splitname=regexp(ratio_id,'_','all');
      |     ratioId=insertBefore(ratio_id,Splitname(end),'5');
      |     eval([char(ratioId), '= 0;']);
      |     set_param([ratioid_b5{n}],'Value',ratioId);
      | 
      |     Splitname=regexp(ratio_id,'_','all');
      |     ratioId=insertBefore(ratio_id,Splitname(end),'6');
      |     eval([char(ratioId), '= 0;']);
      |     set_param([ratioid_b6{n}],'Value',ratioId);
      |     
      |     Splitname=regexp(ratio_id,'_','all');
      |     ratioId=insertBefore(ratio_id,Splitname(end),'7');
      |     eval([char(ratioId), '= 0;']);
      |     set_param([ratioid_b7{n}],'Value',ratioId);
      |     
      |     Splitname=regexp(ratio_id,'_','all');
      |     ratioId=insertBefore(ratio_id,Splitname(end),'8');
      |     eval([char(ratioId), '= 0;']);
      |     set_param([ratioid_b8{n}],'Value',ratioId);
      | end
      | 
      | 
      | % eval([char(RatioId), '_1 = 0;']);
      | % eval([char(RatioId), '_2 = 0;']);
      | % eval([char(RatioId), '_3 = 0;']);
      | % eval([char(RatioId), '_4 = 0;']);
      | % eval([char(RatioId), '_5 = 0;']);
      | % eval([char(RatioId), '_6 = 0;']);
      | % eval([char(RatioId), '_7 = 0;']);
      | % eval([char(RatioId), '_8 = 0;']);
      | % 
      | % 
      | % ratioid_b1 = find_system(gcb,'LookUnderMasks','all','FollowLinks','on','Name','RatioId_block1');
      | % ratioid_b2 = find_system(gcb,'LookUnderMasks','all','FollowLinks','on','Name','RatioId_block2');
      | % ratioid_b3 = find_system(gcb,'LookUnderMasks','all','FollowLinks','on','Name','RatioId_block3');
      | % ratioid_b4 = find_system(gcb,'LookUnderMasks','all','FollowLinks','on','Name','RatioId_block4');
      | % ratioid_b5 = find_system(gcb,'LookUnderMasks','all','FollowLinks','on','Name','RatioId_block5');
      | % ratioid_b6 = find_system(gcb,'LookUnderMasks','all','FollowLinks','on','Name','RatioId_block6');
      | % ratioid_b7 = find_system(gcb,'LookUnderMasks','all','FollowLinks','on','Name','RatioId_block7');
      | % ratioid_b8 = find_system(gcb,'LookUnderMasks','all','FollowLinks','on','Name','RatioId_block8');
      | % 
      | % % 3sets(FaultDetect/DenLock/DenRelease)
      | % for n = 1:length(ratioid_b1)
      | %     set_param([ratioid_b1{n}],'Value',[char(RatioId) '_1']);
      | %     set_param([ratioid_b2{n}],'Value',[char(RatioId) '_2']);
      | %     set_param([ratioid_b3{n}],'Value',[char(RatioId) '_3']);
      | %     set_param([ratioid_b4{n}],'Value',[char(RatioId) '_4']);
      | %     set_param([ratioid_b5{n}],'Value',[char(RatioId) '_5']);
      | %     set_param([ratioid_b6{n}],'Value',[char(RatioId) '_6']);
      | %     set_param([ratioid_b7{n}],'Value',[char(RatioId) '_7']);
      | %     set_param([ratioid_b8{n}],'Value',[char(RatioId) '_8']);
      | % end
      settings: AttributesFormatString=%<MaskType>\nRatioId : = %<RatioId>
      mask Display:
      | % dgn_mask = ['Diagnosis name: ' char(DiagName) '\n Ratio ID: ' char(RatioId) ];
      | dgn_mask = ['Ratio ID: ' char(RatioId) ];
      | 
      | disp(dgn_mask);
      | port_label('input',1,'denlock_status');
      | port_label('input',2,'faultdetect_trigger');
      | 
      | plot([5,5,5])
      | plot([6,6,6])
  AEMS_DEM_REP_IUMPR_DEN_RELEASE_1D : Subsystem  Tag=[LIB]  mask(AEMS_DEM_REP_IUMPR_DEN_RELEASE_1D){RatioId=Dem_RatioId_XXX}
      mask prompts: RatioId "RatioId :"
      mask init:
      | eval([char(RatioId), ' = 0;']);
      | set_param([gcb '/Dem_RepIUMPRDenRelease_call/RatioId_block1'],'Value',char(RatioId));
      | 
      | % ratioid_b1 = find_system(gcb,'LookUnderMasks','all','FollowLinks','on','Name','RatioId_block1');
      | % 
      | % % 3sets(FaultDetect/DenLock/DenRelease)
      | % for n = 1:length(ratioid_b1)
      | %     set_param([ratioid_b1{n}],'Value',char(RatioId));
      | % end
      settings: AttributesFormatString=%<MaskType>\nRatioId : = %<RatioId>
      mask Display:
      | % dgn_mask = ['Diagnosis name: ' char(DiagName) '\n Ratio ID: ' char(RatioId) ];
      | dgn_mask = ['Ratio ID: ' char(RatioId) ];
      | disp(dgn_mask);
      | port_label('input',1,'denlock_status');
      | 
      | plot([5,5,5])
      | plot([6,6,6])
  AEMS_DEM_REP_IUMPR_DEN_RELEASE_2D : Subsystem  Tag=[LIB]  mask(AEMS_DEM_REP_IUMPR_DEN_RELEASE_2D){RatioId=Dem_RatioId_XXX}
      mask prompts: RatioId "RatioId :"
      mask init:
      | lib_path = gcb;
      | Ratio_Id=get_param(lib_path,'RatioId');
      | eval([char(Ratio_Id), '= 0;']);
      | set_param([lib_path '/Dem_RepIUMPRDenRelease_call1/RatioId_block1'],'Value',char(RatioId));
      | Splitname=regexp(Ratio_Id,'_','all');
      | New_RatioId=insertBefore(Ratio_Id,Splitname(end),num2str(2));
      | eval([char(New_RatioId), '= 0;']);
      | set_param([lib_path '/Dem_RepIUMPRDenRelease_call2/RatioId_block2'],'Value',char(New_RatioId));
      | 
      | % eval([char(RatioId), '_1 = 0;']);
      | % eval([char(RatioId), '_2 = 0;']);
      | 
      | % ratioid_b1 = find_system(gcb,'LookUnderMasks','all','FollowLinks','on','Name','RatioId_block1');
      | % ratioid_b2 = find_system(gcb,'LookUnderMasks','all','FollowLinks','on','Name','RatioId_block2');
      | % 
      | % % 3sets(FaultDetect/DenLock/DenRelease)
      | % for n = 1:length(ratioid_b1)
      | %     set_param([ratioid_b1{n}],'Value',[char(RatioId) '_1']);
      | %     set_param([ratioid_b2{n}],'Value',[char(RatioId) '_2']);
      | % end
      settings: AttributesFormatString=%<MaskType>\nRatioId : = %<RatioId>
      mask Display:
      | % dgn_mask = ['Diagnosis name: ' char(DiagName) '\n Ratio ID: ' char(RatioId) ];
      | dgn_mask = ['Ratio ID: ' char(RatioId) ];
      | 
      | disp(dgn_mask);
      | port_label('input',1,'denlock_status');
      | 
      | plot([5,5,5])
      | plot([6,6,6])
  AEMS_DEM_REP_IUMPR_DEN_RELEASE_8D : Subsystem  Tag=[LIB]  mask(AEMS_DEM_REP_IUMPR_DEN_RELEASE_8D){RatioId=Dem_RatioId_XXX}
      mask prompts: RatioId "RatioId :"
      mask init:
      | lib_path=gcb;
      | Ratio_Id=get_param(lib_path,'RatioId');
      | eval([char(Ratio_Id), '= 0;']);
      | set_param([lib_path '/Dem_RepIUMPRDenRelease_call1/RatioId_block1'],'Value',char(RatioId));
      | Splitname=regexp(Ratio_Id,'_','all');
      | 
      | New_RatioId=insertBefore(Ratio_Id,Splitname(end),num2str(2));
      | eval([char(New_RatioId), '= 0;']);
      | set_param([lib_path '/Dem_RepIUMPRDenRelease_call2/RatioId_block2'],'Value',char(New_RatioId));
      | New_RatioId=insertBefore(Ratio_Id,Splitname(end),num2str(3));
      | eval([char(New_RatioId), '= 0;']);
      | set_param([lib_path '/Dem_RepIUMPRDenRelease_call3/RatioId_block3'],'Value',char(New_RatioId));
      | New_RatioId=insertBefore(Ratio_Id,Splitname(end),num2str(4));
      | eval([char(New_RatioId), '= 0;']);
      | set_param([lib_path '/Dem_RepIUMPRDenRelease_call4/RatioId_block4'],'Value',char(New_RatioId));
      | New_RatioId=insertBefore(Ratio_Id,Splitname(end),num2str(5));
      | eval([char(New_RatioId), '= 0;']);
      | set_param([lib_path '/Dem_RepIUMPRDenRelease_call5/RatioId_block5'],'Value',char(New_RatioId));
      | New_RatioId=insertBefore(Ratio_Id,Splitname(end),num2str(6));
      | eval([char(New_RatioId), '= 0;']);
      | set_param([lib_path '/Dem_RepIUMPRDenRelease_call6/RatioId_block6'],'Value',char(New_RatioId));
      | New_RatioId=insertBefore(Ratio_Id,Splitname(end),num2str(7));
      | eval([char(New_RatioId), '= 0;']);
      | set_param([lib_path '/Dem_RepIUMPRDenRelease_call7/RatioId_block7'],'Value',char(New_RatioId));
      | New_RatioId=insertBefore(Ratio_Id,Splitname(end),num2str(8));
      | eval([char(New_RatioId), '= 0;']);
      | set_param([lib_path '/Dem_RepIUMPRDenRelease_call8/RatioId_block8'],'Value',char(New_RatioId));
      | 
      | % % 3sets(FaultDetect/DenLock/DenRelease)
      | % for n = 1:length(ratioid_b1)
      | %     set_param([ratioid_b1{n}],'Value',[char(RatioId) '_1']);
      | %     set_param([ratioid_b2{n}],'Value',[char(RatioId) '_2']);
      | %     set_param([ratioid_b3{n}],'Value',[char(RatioId) '_3']);
      | %     set_param([ratioid_b4{n}],'Value',[char(RatioId) '_4']);
      | %     set_param([ratioid_b5{n}],'Value',[char(RatioId) '_5']);
      | %     set_param([ratioid_b6{n}],'Value',[char(RatioId) '_6']);
      | %     set_param([ratioid_b7{n}],'Value',[char(RatioId) '_7']);
      | %     set_param([ratioid_b8{n}],'Value',[char(RatioId) '_8']);
      | % end
      settings: AttributesFormatString=%<MaskType>\nRatioId : = %<RatioId>
      mask Display:
      | % dgn_mask = ['Diagnosis name: ' char(DiagName) '\n Ratio ID: ' char(RatioId) ];
      | dgn_mask = ['Ratio ID: ' char(RatioId) ];
      | 
      | disp(dgn_mask);
      | port_label('input',1,'denlock_status');
      | 
      | plot([5,5,5])
      | plot([6,6,6])
  AEMS_DEM_REP_IUMPR_FAULTDETECT_1D : Subsystem  Tag=[LIB]  mask(AEMS_DEM_REP_IUMPR_FAULTDETECT_1D){RatioId=Dem_RatioId_XXX}
      mask prompts: RatioId "RatioId :"
      mask init: same as AEMS_Standard_Library/SUB/AEMS_DEM_REP_IUMPR_1D
      settings: AttributesFormatString=%<MaskType>\nRatioId : = %<RatioId>
      mask Display:
      | % dgn_mask = ['Diagnosis name: ' char(DiagName) '\n Ratio ID: ' char(RatioId) ];
      | dgn_mask = ['Ratio ID: ' char(RatioId) ];
      | disp(dgn_mask);
      | port_label('input',1,'faultdetect_trigger');
      | 
      | plot([5,5,5])
      | plot([6,6,6])
  AEMS_DEM_REP_IUMPR_FAULTDETECT_2D : Subsystem  Tag=[LIB]  mask(AEMS_DEM_REP_IUMPR_FAULTDETECT_2D){RatioId=Dem_RatioId_XXX}
      mask prompts: RatioId "RatioId :"
      mask init:
      | % eval([char(RatioId), '_1 = 0;']);
      | % eval([char(RatioId), '_2 = 0;']);
      | 
      | % ratioid_b1 = find_system(gcb,'LookUnderMasks','all','FollowLinks','on','Name','RatioId_block1');
      | % ratioid_b2 = find_system(gcb,'LookUnderMasks','all','FollowLinks','on','Name','RatioId_block2');
      | % 
      | % % 3sets(FaultDetect/DenLock/DenRelease)
      | % for n = 1:length(ratioid_b1)
      | %     set_param([ratioid_b1{n}],'Value',[char(RatioId) '_1']);
      | %     set_param([ratioid_b2{n}],'Value',[char(RatioId) '_2']);
      | % end
      | 
      | lib_path = gcb;
      | 
      | Ratio_Id=get_param(lib_path,'RatioId');
      | ratioid_b = find_system(lib_path,'LookUnderMasks','all','FollowLinks','on','regexp','on','Name','^RatioId_block');
      | ratioid_b1 = find_system(lib_path,'LookUnderMasks','all','FollowLinks','on','Name','RatioId_block1');
      | eval([char(Ratio_Id), '= 0;']);
      | set_param([ratioid_b1{:}],'Value',char(Ratio_Id));
      | 
      | Splitname=regexp(Ratio_Id,'_','all');
      | New_RatioId=insertBefore(Ratio_Id,Splitname(end),num2str(2));
      | eval([char(New_RatioId), '= 0;']);
      | set_param([ratioid_b{2}],'Value',char(New_RatioId));
      settings: AttributesFormatString=%<MaskType>\nRatioId : = %<RatioId>
      mask Display:
      | % dgn_mask = ['Diagnosis name: ' char(DiagName) '\n Ratio ID: ' char(RatioId) ];
      | dgn_mask = ['Ratio ID: ' char(RatioId) ];
      | 
      | disp(dgn_mask);
      | port_label('input',1,'faultdetect_trigger');
      | 
      | plot([5,5,5])
      | plot([6,6,6])
  AEMS_DEM_REP_IUMPR_FAULTDETECT_8D : Subsystem  Tag=[LIB]  mask(AEMS_DEM_REP_IUMPR_FAULTDETECT_8D){RatioId=Dem_RatioId_XXX}
      mask prompts: RatioId "RatioId :"
      mask init:
      | % eval([char(RatioId), '_1 = 0;']);
      | % eval([char(RatioId), '_2 = 0;']);
      | % eval([char(RatioId), '_3 = 0;']);
      | % eval([char(RatioId), '_4 = 0;']);
      | % eval([char(RatioId), '_5 = 0;']);
      | % eval([char(RatioId), '_6 = 0;']);
      | % eval([char(RatioId), '_7 = 0;']);
      | % eval([char(RatioId), '_8 = 0;']);
      | 
      | lib_path = gcb;
      | 
      | Ratio_Id=get_param(lib_path,'RatioId');
      | ratioid_b = find_system(lib_path,'LookUnderMasks','all','FollowLinks','on','regexp','on','Name','^RatioId_block');
      | ratioid_b1 = find_system(lib_path,'LookUnderMasks','all','FollowLinks','on','Name','RatioId_block1');
      | eval([char(Ratio_Id), ' = 0;']);
      | set_param([ratioid_b1{:}],'Value',char(Ratio_Id));
      | 
      | for len=2:length(ratioid_b)
      | Splitname=regexp(Ratio_Id,'_','all');
      | New_RatioId=insertBefore(Ratio_Id,Splitname(end),num2str(len));
      | eval([char(New_RatioId), ' = 0;']);
      | set_param([ratioid_b{len}],'Value',char(New_RatioId));
      | end
      | 
      | % ratioid_b1 = find_system(gcb,'LookUnderMasks','all','FollowLinks','on','Name','RatioId_block1');
      | % ratioid_b2 = find_system(gcb,'LookUnderMasks','all','FollowLinks','on','Name','RatioId_block2');
      | % ratioid_b3 = find_system(gcb,'LookUnderMasks','all','FollowLinks','on','Name','RatioId_block3');
      | % ratioid_b4 = find_system(gcb,'LookUnderMasks','all','FollowLinks','on','Name','RatioId_block4');
      | % ratioid_b5 = find_system(gcb,'LookUnderMasks','all','FollowLinks','on','Name','RatioId_block5');
      | % ratioid_b6 = find_system(gcb,'LookUnderMasks','all','FollowLinks','on','Name','RatioId_block6');
      | % ratioid_b7 = find_system(gcb,'LookUnderMasks','all','FollowLinks','on','Name','RatioId_block7');
      | % ratioid_b8 = find_system(gcb,'LookUnderMasks','all','FollowLinks','on','Name','RatioId_block8');
      | % 
      | % % 3sets(FaultDetect/DenLock/DenRelease)
      | % for n = 1:length(ratioid_b1)
      | %     set_param([ratioid_b1{n}],'Value',[char(RatioId) '_1']);
      | %     set_param([ratioid_b2{n}],'Value',[char(RatioId) '_2']);
      | %     set_param([ratioid_b3{n}],'Value',[char(RatioId) '_3']);
      | %     set_param([ratioid_b4{n}],'Value',[char(RatioId) '_4']);
      | %     set_param([ratioid_b5{n}],'Value',[char(RatioId) '_5']);
      | %     set_param([ratioid_b6{n}],'Value',[char(RatioId) '_6']);
      | %     set_param([ratioid_b7{n}],'Value',[char(RatioId) '_7']);
      | %     set_param([ratioid_b8{n}],'Value',[char(RatioId) '_8']);
      | % end
      settings: AttributesFormatString=%<MaskType>\nRatioId : = %<RatioId>
      mask Display:
      | % dgn_mask = ['Diagnosis name: ' char(DiagName) '\n Ratio ID: ' char(RatioId) ];
      | dgn_mask = ['Ratio ID: ' char(RatioId) ];
      | 
      | disp(dgn_mask);
      | port_label('input',1,'faultdetect_trigger');
      | 
      | plot([5,5,5])
      | plot([6,6,6])
  AEMS_DEM_SETDTR : Subsystem  Tag=[LIB]  mask(AEMS_DEM_SETDTR){}
      mask help:
      | This library calls AUTOSAR standard functions.
      | To know more details, please refer AUTOSAR DEM00765.
      settings: AttributesFormatString=%<MaskType>
      mask Display:
      | disp(['Dem_SetDTR \n \n \n \n \n']);
      | plot([5,5,5])
      | plot([6,6,6])
      | port_label('input',1,'DTRId')
      | port_label('input',2,'TestResult')
      | port_label('input',3,'LowerLimit')
      | port_label('input',4,'UpperLimit')
      | port_label('input',5,'Ctrlval')
  AEMS_DEM_SETENABLECONDITION : Subsystem  Tag=[LIB]  mask(AEMS_DEM_SETENABLECONDITION){}
      mask help:
      | This library calls AUTOSAR standard functions.
      | To know more details, please refer AUTOSAR DEM00201.
      settings: AttributesFormatString=%<MaskType>
      mask Display:
      | disp(['Dem_SetEnableCondition']);
      | plot([5,5,5])
      | plot([6,6,6])
      | 
      | port_label('input',1,'EnableConditionID');
      | port_label('input',2,'ConditionFulfilled');
  AEMS_DEM_SETEVENTAVAILABLE : Subsystem  Tag=[LIB]  mask(AEMS_DEM_SETEVENTAVAILABLE){}
      mask help:
      | This library calls AUTOSAR standard functions.
      | To know more details, please refer AUTOSAR DEM01080.
      settings: AttributesFormatString=%<MaskType>
      mask Display:
      | disp(['Dem_SetEventAvailable \n \n \n \n \n']);
      | plot([5,5,5])
      | plot([6,6,6])
      | port_label('input',1,'EventId')
      | port_label('input',2,'AvailableStatus')
      | %port_label('output',1,'Dem_Result')
  AEMS_DEM_SETEVENTDISABLED : Subsystem  Tag=[LIB]  mask(AEMS_DEM_SETEVENTDISABLED){}
      mask help:
      | This library calls AUTOSAR standard functions.
      | To know more details, please refer AUTOSAR DEM00312.
      settings: AttributesFormatString=%<MaskType>
      mask Display:
      | disp(['Dem_SetEventDisabled \n \n \n \n \n']);
      | plot([5,5,5])
      | plot([6,6,6])
      | port_label('input',1,'EventId')
  AEMS_DEM_SETEVENTSTATUS : Subsystem  Tag=[LIB]  mask(AEMS_DEM_SETEVENTSTATUS){}
      mask help:
      | This library calls AUTOSAR standard functions.
      | To know more details, please refer AUTOSAR DEM00183.
      settings: AttributesFormatString=%<MaskType>
      mask Display:
      | disp(['Dem_SetEventStatus \n \n \n \n \n']);
      | plot([5,5,5])
      | plot([6,6,6])
      | port_label('input',1,'EventId')
      | port_label('input',2,'EventStatus')
      | %port_label('output',1,'Dem_Result')
  AEMS_DEM_SETIUMPRDENCONDITION : Subsystem  Tag=[LIB]  mask(AEMS_DEM_SETIUMPRDENCONDITION){}
      mask help:
      | This library calls AUTOSAR standard functions.
      | To know more details, please refer AUTOSAR DEM00733.
      settings: AttributesFormatString=%<MaskType>
      mask Display:
      | disp(['Dem_SetIUMPRDenCondition \n \n \n \n \n']);
      | plot([5,5,5])
      | plot([6,6,6])
      | port_label('input',1,'ConditionId')
      | port_label('input',2,'ConditionStatus')
      | %port_label('output',1,'Dem_Result')
  AEMS_DEM_SETOPERATIONCYCLESTATE : Subsystem  Tag=[LIB]  mask(AEMS_DEM_SETOPERATIONCYCLESTATE){}
      mask help:
      | This library calls AUTOSAR standard functions.
      | To know more details, please refer AUTOSAR DEM00194.
      settings: AttributesFormatString=%<MaskType>
      mask Display:
      | disp(['Dem_SetOperationCycleState \n \n \n \n \n']);
      | plot([5,5,5])
      | plot([6,6,6])
      | port_label('input',1,'OperationCycleId')
      | port_label('input',2,'CycleState')
      | %port_label('output',1,'Dem_Result')
  AEMS_DEM_SETPFCCYCLEQUALIFIED : Subsystem  Tag=[LIB]  mask(AEMS_DEM_SETPFCCYCLEQUALIFIED){}
      mask help:
      | This library calls AUTOSAR standard functions.
      | To know more details, please refer AUTOSAR DEM00739.
      settings: AttributesFormatString=%<MaskType>
      mask Display:
      | disp(['Dem_SetPfcCycleQualified \n \n \n \n \n']);
      | plot([5,5,5])
      | plot([6,6,6])
  AEMS_DEM_SETSTORAGECONDITION : Subsystem  Tag=[LIB]  mask(AEMS_DEM_SETSTORAGECONDITION){}
      mask help:
      | This library calls AUTOSAR standard functions.
      | To know more details, please refer AUTOSAR [SWS_Dem_00556].
      settings: AttributesFormatString=%<MaskType>
      mask Display:
      | disp(['Dem_SetStorageCondition']);
      | plot([5,5,5])
      | plot([6,6,6])
      | 
      | port_label('input',1,'StorageConditionID,');
      | port_label('input',2,'ConditionFulfilled');
  AEMS_DEM_SET_DTR_1DS : Subsystem  Tag=[LIB]  mask(AEMS_DEM_SET_DTR_1DS){conv_type=0x01, EventId=Dem_DtrId_XXX, resol=1, dlim=0, ulim=65535}
      mask prompts: conv_type "Conversion Type :"; EventId "EventId :"; resol "resolution"; dlim "lowerlimit"; ulim "upperlimit"
      mask init:
      | eval([char(EventId) '= 0;']);
      | % eval([char(DtrId) '= 0;']);
      | % eval([char(Ctrlval) '= 0;']);
      | eval(['DEM_DTR_CTL_NORMAL = 0;']);
      | eval(['DEM_DTR_CTL_INVISIBLE = 4;']);
      | 
      | 
      | dtrid_b1 = find_system(gcb,'LookUnderMasks','all','FollowLinks','on','Name','DTRId_block');
      | % ctrlval_b1 = find_system(gcb,'LookUnderMasks','all','FollowLinks','on','Name','Ctrlval_block');
      | resol_b1 = find_system(gcb,'LookUnderMasks','all','FollowLinks','on','Name','resolution_block1');
      | resol_b2 = find_system(gcb,'LookUnderMasks','all','FollowLinks','on','Name','resolution_block2');
      | 
      | resol_b3 = find_system(gcb,'LookUnderMasks','all','FollowLinks','on','Name','Resolution_block1');
      | resol_b4 = find_system(gcb,'LookUnderMasks','all','FollowLinks','on','Name','Resolution_block2');
      | resol_b5 = find_system(gcb,'LookUnderMasks','all','FollowLinks','on','Name','Resolution_block3');
      | 
      | limit_b1 = find_system(gcb,'LookUnderMasks','all','FollowLinks','on','Name','Limitter1');
      | limit_b2 = find_system(gcb,'LookUnderMasks','all','FollowLinks','on','Name','Limitter2');
      | limit_b3 = find_system(gcb,'LookUnderMasks','all','FollowLinks','on','Name','Limitter3');
      | 
      | 
      | for n = 1:length(dtrid_b1)
      |     set_param([dtrid_b1{n}],'Value',[char(EventId)]);
      | end
      | 
      | % for n = 1:length(ctrlval_b1)
      | %     set_param([ctrlval_b1{n}],'Value',[char(Ctrlval)]);
      | % end
      | 
      | set_param([resol_b1{:}],'Value',resol);
      | set_param([resol_b2{:}],'Value',resol);
      | set_param([resol_b3{:}],'Value',resol);
      | set_param([resol_b4{:}],'Value',resol);
      | set_param([resol_b5{:}],'Value',resol);
      | 
      | set_param([limit_b1{:}],'UpperLimit',ulim);
      | set_param([limit_b2{:}],'UpperLimit',ulim);
      | set_param([limit_b3{:}],'UpperLimit',ulim);
      | 
      | set_param([limit_b1{:}],'LowerLimit',dlim);
      | set_param([limit_b2{:}],'LowerLimit',dlim);
      | set_param([limit_b3{:}],'LowerLimit',dlim);
      settings: AttributesFormatString=%<MaskType>\nConversion Type : = %<conv_type>\nEventId : = %<EventId>\nresolution = %<resol>\nlowerlimit = %<dlim>\nupperlimit = %<ulim>
      mask TypeOptions conv_type: 0x01 | 0x02 | 0x03 | 0x04 | 0x05 | 0x06 | 0x07 | 0x08 | 0x09 | 0x0A | 0x0B | 0x0C | 0x0D | 0x0E | 0x0F | 0x10 | 0x11 | 0x12 | 0x13 | 0x14 | 0x15 | 0x16 | 0x17 | 0x18 | 0x19 | 0x1A | 0x1B | 0x1C | 0x1D | 0x1E | 0x1F | 0x20 | 0x21 | 0x22 | 0x23 | 0x24 | 0x25 | 0x26 | 0x27 | 0x28 | 0x29 | 0x2A | 0x2B | 0x2C | 0x2D | 0x2E | 0x2F | 0x30 | 0x31 | 0x32 | 0x33 | 0x34 | 0x35 | 0x36 | 0x37 | 0x38 | 0x39 | 0x3A | 0x3B | 0x3C | 0x3D | 0x3E | 0x3F | 0x40 | 0x41 | 0x42 | 0x43 | 0x44 | 0x81 | 0x82 | 0x83 | 0x84 | 0x85 | 0x86 | 0x87 | 0x8A | 0x8B | 0x8C | 0x8D | 0x8E | 0x8F | 0x90 | 0x91 | 0x92 | 0x96 | 0x97 | 0x98 | 0x99 | 0x9C | 0x9D | 0xA8 | 0xA9 | 0xAD | 0xAE | 0xAF | 0xB0 | 0xB1 | 0xFA | 0xFB | 0xFC | 0xFD | 0xFE
      mask Display:
      | port_label('input',1,'set_flag');
      | port_label('input',2,'testresult');
      | port_label('input',3,'lowerlimit');
      | port_label('input',4,'upperlimit');
      | port_label('input',5,'ctrl_flag');
      | 
      | dgn_mask = [char(EventId) '\n Conversion : ' conv_type];
      | 
      | disp(dgn_mask);
      | plot([5,5,5])
      | plot([6,6,6])
  AEMS_DEM_SET_DTR_1DU : Subsystem  Tag=[LIB]  mask(AEMS_DEM_SET_DTR_1DU){conv_type=0x24, EventId=Dem_DtrId_XXX, resol=1, dlim=0, ulim=1}
      mask prompts: conv_type "Conversion Type :"; resol "resolution"; dlim "lowerlimit"; ulim "upperlimit"
      mask init:
      | eval([char(EventId) '= 0;']);
      | % eval([char(DtrId) '= 0;']);
      | % eval([char(Ctrlval) '= 0;']);
      | eval(['DEM_DTR_CTL_NORMAL = 0;']);
      | eval(['DEM_DTR_CTL_INVISIBLE = 4;']);
      | 
      | dtrid_b1 = find_system(gcb,'LookUnderMasks','all','FollowLinks','on','Name','DTRId_block');
      | % ctrlval_b1 = find_system(gcb,'LookUnderMasks','all','FollowLinks','on','Name','Ctrlval_block');
      | %offsetblock is not been set. Please add if requested.
      | limit_b1 = find_system(gcb,'LookUnderMasks','all','FollowLinks','on','Name','Limitter1');
      | limit_b2 = find_system(gcb,'LookUnderMasks','all','FollowLinks','on','Name','Limitter2');
      | limit_b3 = find_system(gcb,'LookUnderMasks','all','FollowLinks','on','Name','Limitter3');
      | 
      | for n = 1:length(dtrid_b1)
      |     set_param([dtrid_b1{n}],'Value',[char(EventId)]);
      | end
      | 
      | % for n = 1:length(ctrlval_b1)
      | %     set_param([ctrlval_b1{n}],'Value',[char(Ctrlval)]);
      | % end
      | 
      | set_param([limit_b1{:}],'UpperLimit',ulim);
      | set_param([limit_b2{:}],'UpperLimit',ulim);
      | set_param([limit_b3{:}],'UpperLimit',ulim);
      | 
      | set_param([limit_b1{:}],'LowerLimit',dlim);
      | set_param([limit_b2{:}],'LowerLimit',dlim);
      | set_param([limit_b3{:}],'LowerLimit',dlim);
      settings: AttributesFormatString=%<MaskType>\nConversion Type : = %<conv_type>\nEventId = %<EventId>\nresolution = %<resol>\nlowerlimit = %<dlim>\nupperlimit = %<ulim>
      mask TypeOptions conv_type: 0x01 | 0x02 | 0x03 | 0x04 | 0x05 | 0x06 | 0x07 | 0x08 | 0x09 | 0x0A | 0x0B | 0x0C | 0x0D | 0x0E | 0x0F | 0x10 | 0x11 | 0x12 | 0x13 | 0x14 | 0x15 | 0x16 | 0x17 | 0x18 | 0x19 | 0x1A | 0x1B | 0x1C | 0x1D | 0x1E | 0x1F | 0x20 | 0x21 | 0x22 | 0x23 | 0x24 | 0x25 | 0x26 | 0x27 | 0x28 | 0x29 | 0x2A | 0x2B | 0x2C | 0x2D | 0x2E | 0x2F | 0x30 | 0x31 | 0x32 | 0x33 | 0x34 | 0x35 | 0x36 | 0x37 | 0x38 | 0x39 | 0x3A | 0x3B | 0x3C | 0x3D | 0x3E | 0x3F | 0x40 | 0x41 | 0x42 | 0x43 | 0x44 | 0x81 | 0x82 | 0x83 | 0x84 | 0x85 | 0x86 | 0x87 | 0x8A | 0x8B | 0x8C | 0x8D | 0x8E | 0x8F | 0x90 | 0x91 | 0x92 | 0x96 | 0x97 | 0x98 | 0x99 | 0x9C | 0x9D | 0xA8 | 0xA9 | 0xAD | 0xAE | 0xAF | 0xB0 | 0xB1 | 0xFA | 0xFB | 0xFC | 0xFDC | 0xFE
      mask Display:
      | port_label('input',1,'set_flag');
      | port_label('input',2,'testresult');
      | port_label('input',3,'lowerlimit');
      | port_label('input',4,'upperlimit');
      | port_label('input',5,'ctrl_flag');
      | 
      | dgn_mask = [char(EventId) '\n Conversion : ' conv_type];
      | 
      | disp(dgn_mask);
      | 
      | plot([5,5,5])
      | plot([6,6,6])
  AEMS_DEM_SET_DTR_2DS : Subsystem  Tag=[LIB]  mask(AEMS_DEM_SET_DTR_2DS){conv_type=0x01, EventId=Dem_DtrId_XXX, resol=1, dlim=0, ulim=1}
      mask prompts: conv_type "Conversion Type :"; EventId "EventId :"; resol "resolution"; dlim "lowerlimit"; ulim "upperlimit"
      mask init:
      | % eval([char(EventId) '_1 = 0;']);
      | % eval([char(EventId) '_2 = 0;']);
      | % eval([char(Ctrlval) '_1 = 0;']);
      | % eval([char(Ctrlval) '_2 = 0;']);
      | eval(['DEM_DTR_CTL_NORMAL = 0;']);
      | eval(['DEM_DTR_CTL_INVISIBLE = 4;']);
      | 
      | Event_Id=get_param(gcb,'EventId');
      | 
      | dtrid_b1 = find_system(gcb,'LookUnderMasks','all','FollowLinks','on','Name','DTRId_block1');
      | eval([char(Event_Id) '= 0;']);
      | set_param(dtrid_b1{:},'Value',char(Event_Id));
      | 
      | dtrid_b2 = find_system(gcb,'LookUnderMasks','all','FollowLinks','on','Name','DTRId_block2');
      | Splitname=regexp(Event_Id,'_','all');
      | New_EventId=insertBefore(Event_Id,Splitname(end),num2str(2));
      | eval([char(New_EventId) '= 0;']);
      | set_param(dtrid_b2{:},'Value',char(New_EventId));
      | 
      | resol_b1 = find_system(gcb,'LookUnderMasks','all','FollowLinks','on','Name','resolution_block1');
      | resol_b2 = find_system(gcb,'LookUnderMasks','all','FollowLinks','on','Name','resolution_block2');
      | 
      | % dtrid_b1 = find_system(gcb,'LookUnderMasks','all','FollowLinks','on','Name','DTRId_block1');
      | % dtrid_b2 = find_system(gcb,'LookUnderMasks','all','FollowLinks','on','Name','DTRId_block2');
      | 
      | % ctrlval_b1 = find_system(gcb,'LookUnderMasks','all','FollowLinks','on','Name','Ctrlval_block1');
      | % ctrlval_b2 = find_system(gcb,'LookUnderMasks','all','FollowLinks','on','Name','Ctrlval_block2');
      | 
      | resol_b3 = find_system(gcb,'LookUnderMasks','all','FollowLinks','on','Name','Resolution_block1');
      | resol_b4 = find_system(gcb,'LookUnderMasks','all','FollowLinks','on','Name','Resolution_block2');
      | resol_b5 = find_system(gcb,'LookUnderMasks','all','FollowLinks','on','Name','Resolution_block3');
      | resol_b6 = find_system(gcb,'LookUnderMasks','all','FollowLinks','on','Name','Resolution_block4');
      | resol_b7 = find_system(gcb,'LookUnderMasks','all','FollowLinks','on','Name','Resolution_block5');
      | resol_b8 = find_system(gcb,'LookUnderMasks','all','FollowLinks','on','Name','Resolution_block6');
      | 
      | limit_b1 = find_system(gcb,'LookUnderMasks','all','FollowLinks','on','Name','Limitter1');
      | limit_b2 = find_system(gcb,'LookUnderMasks','all','FollowLinks','on','Name','Limitter2');
      | limit_b3 = find_system(gcb,'LookUnderMasks','all','FollowLinks','on','Name','Limitter3');
      | limit_b4 = find_system(gcb,'LookUnderMasks','all','FollowLinks','on','Name','Limitter4');
      | limit_b5 = find_system(gcb,'LookUnderMasks','all','FollowLinks','on','Name','Limitter5');
      | limit_b6 = find_system(gcb,'LookUnderMasks','all','FollowLinks','on','Name','Limitter6');
      | 
      | % for n = 1:length(ctrlval_b1)
      | %     set_param([ctrlval_b1{n}],'Value',[char(Ctrlval) '_1']);
      | %     set_param([ctrlval_b2{n}],'Value',[char(Ctrlval) '_2']);
      | % end
      | 
      | set_param([resol_b1{:}],'Value',resol);
      | set_param([resol_b2{:}],'Value',resol);
      | set_param([resol_b3{:}],'Value',resol);
      | set_param([resol_b4{:}],'Value',resol);
      | set_param([resol_b5{:}],'Value',resol);
      | set_param([resol_b6{:}],'Value',resol);
      | set_param([resol_b7{:}],'Value',resol);
      | set_param([resol_b8{:}],'Value',resol);
      | 
      | set_param([limit_b1{:}],'UpperLimit',ulim);
      | set_param([limit_b2{:}],'UpperLimit',ulim);
      | set_param([limit_b3{:}],'UpperLimit',ulim);
      | set_param([limit_b4{:}],'UpperLimit',ulim);
      | set_param([limit_b5{:}],'UpperLimit',ulim);
      | set_param([limit_b6{:}],'UpperLimit',ulim);
      |  
      | set_param([limit_b1{:}],'LowerLimit',dlim);
      | set_param([limit_b2{:}],'LowerLimit',dlim);
      | set_param([limit_b3{:}],'LowerLimit',dlim);
      | set_param([limit_b4{:}],'LowerLimit',dlim);
      | set_param([limit_b5{:}],'LowerLimit',dlim);
      | set_param([limit_b6{:}],'LowerLimit',dlim);
      settings: AttributesFormatString=%<MaskType>\nConversion Type : = %<conv_type>\nEventId : = %<EventId>\nresolution = %<resol>\nlowerlimit = %<dlim>\nupperlimit = %<ulim>
      mask TypeOptions conv_type: 0x01 | 0x02 | 0x03 | 0x04 | 0x05 | 0x06 | 0x07 | 0x08 | 0x09 | 0x0A | 0x0B | 0x0C | 0x0D | 0x0E | 0x0F | 0x10 | 0x11 | 0x12 | 0x13 | 0x14 | 0x15 | 0x16 | 0x17 | 0x18 | 0x19 | 0x1A | 0x1B | 0x1C | 0x1D | 0x1E | 0x1F | 0x20 | 0x21 | 0x22 | 0x23 | 0x24 | 0x25 | 0x26 | 0x27 | 0x28 | 0x29 | 0x2A | 0x2B | 0x2C | 0x2D | 0x2E | 0x2F | 0x30 | 0x31 | 0x32 | 0x33 | 0x34 | 0x35 | 0x36 | 0x37 | 0x38 | 0x39 | 0x3A | 0x3B | 0x3C | 0x3D | 0x3E | 0x3F | 0x40 | 0x41 | 0x42 | 0x43 | 0x44 | 0x81 | 0x82 | 0x83 | 0x84 | 0x85 | 0x86 | 0x87 | 0x8A | 0x8B | 0x8C | 0x8D | 0x8E | 0x8F | 0x90 | 0x91 | 0x92 | 0x96 | 0x97 | 0x98 | 0x99 | 0x9C | 0x9D | 0xA8 | 0xA9 | 0xAD | 0xAE | 0xAF | 0xB0 | 0xB1 | 0xFA | 0xFB | 0xFC | 0xFD | 0xFE
      mask Display:
      | port_label('input',1,'set_flag');
      | port_label('input',2,'testresult');
      | port_label('input',3,'lowerlimit');
      | port_label('input',4,'upperlimit');
      | port_label('input',5,'crtl_flag');
      | 
      | dgn_mask = [char(EventId) '\n Conversion : ' conv_type];
      | 
      | disp(dgn_mask);
      | 
      | plot([5,5,5])
      | plot([6,6,6])
  AEMS_DEM_SET_DTR_2DU : Subsystem  Tag=[LIB]  mask(AEMS_DEM_SET_DTR_2DU){conv_type=0x24, EventId=Dem_DtrId_XXX, resol=1, dlim=0, ulim=1}
      mask prompts: conv_type "Conversion Type :"; resol "resolution"; dlim "lowerlimit"; ulim "upperlimit"
      mask init:
      | % eval([char(EventId) '_1 = 0;']);
      | % eval([char(EventId) '_2 = 0;']);
      | % eval([char(Ctrlval) '_1 = 0;']);
      | % eval([char(Ctrlval) '_2 = 0;']);
      | eval(['DEM_DTR_CTL_NORMAL = 0;']);
      | eval(['DEM_DTR_CTL_INVISIBLE = 4;']);
      | 
      | 
      | Event_Id=get_param(gcb,'EventId');
      | 
      | dtrid_b1 = find_system(gcb,'LookUnderMasks','all','FollowLinks','on','Name','DTRId_block1');
      | eval([char(Event_Id) '= 0;']);
      | set_param(dtrid_b1{:},'Value',char(Event_Id));
      | 
      | dtrid_b2 = find_system(gcb,'LookUnderMasks','all','FollowLinks','on','Name','DTRId_block2');
      | Splitname=regexp(Event_Id,'_','all');
      | New_EventId=insertBefore(Event_Id,Splitname(end),num2str(2));
      | eval([char(New_EventId) '= 0;']);
      | set_param(dtrid_b2{:},'Value',char(New_EventId));
      | 
      | 
      | % ctrlval_b1 = find_system(gcb,'LookUnderMasks','all','FollowLinks','on','Name','Ctrlval_block1');
      | % ctrlval_b2 = find_system(gcb,'LookUnderMasks','all','FollowLinks','on','Name','Ctrlval_block2');
      | % offsetblock is not been set. Please add if requested.
      | limit_b1 = find_system(gcb,'LookUnderMasks','all','FollowLinks','on','Name','Limitter1');
      | limit_b2 = find_system(gcb,'LookUnderMasks','all','FollowLinks','on','Name','Limitter2');
      | limit_b3 = find_system(gcb,'LookUnderMasks','all','FollowLinks','on','Name','Limitter3');
      | limit_b4 = find_system(gcb,'LookUnderMasks','all','FollowLinks','on','Name','Limitter4');
      | limit_b5 = find_system(gcb,'LookUnderMasks','all','FollowLinks','on','Name','Limitter5');
      | limit_b6 = find_system(gcb,'LookUnderMasks','all','FollowLinks','on','Name','Limitter6');
      | 
      | % for n = 1:length(dtrid_b1)
      | %     set_param([dtrid_b1{n}],'Value',[char(EventId) '_1']);
      | %     set_param([dtrid_b2{n}],'Value',[char(EventId) '_2']);
      | % end
      | 
      | % for n = 1:length(ctrlval_b1)
      | %     set_param([ctrlval_b1{n}],'Value',[char(Ctrlval) '_1']);
      | %     set_param([ctrlval_b2{n}],'Value',[char(Ctrlval) '_2']);
      | % end
      | 
      | set_param([limit_b1{:}],'UpperLimit',ulim);
      | set_param([limit_b2{:}],'UpperLimit',ulim);
      | set_param([limit_b3{:}],'UpperLimit',ulim);
      | set_param([limit_b4{:}],'UpperLimit',ulim);
      | set_param([limit_b5{:}],'UpperLimit',ulim);
      | set_param([limit_b6{:}],'UpperLimit',ulim);
      | 
      | set_param([limit_b1{:}],'LowerLimit',dlim);
      | set_param([limit_b2{:}],'LowerLimit',dlim);
      | set_param([limit_b3{:}],'LowerLimit',dlim);
      | set_param([limit_b4{:}],'LowerLimit',dlim);
      | set_param([limit_b5{:}],'LowerLimit',dlim);
      | set_param([limit_b6{:}],'LowerLimit',dlim);
      settings: AttributesFormatString=%<MaskType>\nConversion Type : = %<conv_type>\nEventId = %<EventId>\nresolution = %<resol>\nlowerlimit = %<dlim>\nupperlimit = %<ulim>
      mask TypeOptions conv_type: 0x01 | 0x02 | 0x03 | 0x04 | 0x05 | 0x06 | 0x07 | 0x08 | 0x09 | 0x0A | 0x0B | 0x0C | 0x0D | 0x0E | 0x0F | 0x10 | 0x11 | 0x12 | 0x13 | 0x14 | 0x15 | 0x16 | 0x17 | 0x18 | 0x19 | 0x1A | 0x1B | 0x1C | 0x1D | 0x1E | 0x1F | 0x20 | 0x21 | 0x22 | 0x23 | 0x24 | 0x25 | 0x26 | 0x27 | 0x28 | 0x29 | 0x2A | 0x2B | 0x2C | 0x2D | 0x2E | 0x2F | 0x30 | 0x31 | 0x32 | 0x33 | 0x34 | 0x35 | 0x36 | 0x37 | 0x38 | 0x39 | 0x3A | 0x3B | 0x3C | 0x3D | 0x3E | 0x3F | 0x40 | 0x41 | 0x42 | 0x43 | 0x44 | 0x81 | 0x82 | 0x83 | 0x84 | 0x85 | 0x86 | 0x87 | 0x8A | 0x8B | 0x8C | 0x8D | 0x8E | 0x8F | 0x90 | 0x91 | 0x92 | 0x96 | 0x97 | 0x98 | 0x99 | 0x9C | 0x9D | 0xA8 | 0xA9 | 0xAD | 0xAE | 0xAF | 0xB0 | 0xB1 | 0xFA | 0xFB | 0xFC | 0xFD | 0xFE
      mask Display:
      | port_label('input',1,'set_flag');
      | port_label('input',2,'testresult');
      | port_label('input',3,'lowerlimit');
      | port_label('input',4,'upperlimit');
      | port_label('input',5,'ctrl_flag');
      | 
      | dgn_mask = [char(EventId) '\n Conversion : ' conv_type];
      | 
      | disp(dgn_mask);
      | 
      | plot([5,5,5])
      | plot([6,6,6])
  AEMS_DEM_SET_DTR_8DS : Subsystem  Tag=[LIB]  mask(AEMS_DEM_SET_DTR_8DS){conv_type=0x01, EventId=Dem_DtrId_XXX, resol=1, dlim=0, ulim=1}
      mask prompts: conv_type "Conversion Type :"; resol "reslution"; dlim "lowerlimit"; ulim "upperlimit"
      mask init:
      | % eval([char(EventId) '_1 = 0;']);
      | % eval([char(EventId) '_2 = 0;']);
      | % eval([char(EventId) '_3 = 0;']);
      | % eval([char(EventId) '_4 = 0;']);
      | % eval([char(EventId) '_5 = 0;']);
      | % eval([char(EventId) '_6 = 0;']);
      | % eval([char(EventId) '_7 = 0;']);
      | % eval([char(EventId) '_8 = 0;']);
      | % eval([char(Ctrlval) '_1 = 0;']);
      | % eval([char(Ctrlval) '_2 = 0;']);
      | % eval([char(Ctrlval) '_3 = 0;']);
      | % eval([char(Ctrlval) '_4 = 0;']);
      | % eval([char(Ctrlval) '_5 = 0;']);
      | % eval([char(Ctrlval) '_6 = 0;']);
      | % eval([char(Ctrlval) '_7 = 0;']);
      | % eval([char(Ctrlval) '_8 = 0;']);
      | eval(['DEM_DTR_CTL_NORMAL = 0;']);
      | eval(['DEM_DTR_CTL_INVISIBLE = 4;']);
      | 
      | resol_b1 = find_system(gcb,'LookUnderMasks','all','FollowLinks','on','Name','resolution_block1');
      | resol_b2 = find_system(gcb,'LookUnderMasks','all','FollowLinks','on','Name','resolution_block2');
      | 
      | Event_Id=get_param(gcb,'EventId');
      | 
      | dtrid_b1 = find_system(gcb,'LookUnderMasks','all','FollowLinks','on','Name','DTRId_block1');
      | eval([char(Event_Id) '= 0;']);
      | set_param(dtrid_b1{:},'Value',char(Event_Id));
      | 
      | dtrid_b = find_system(gcb,'LookUnderMasks','all','FollowLinks','on','regexp','on','Name','^DTRId_block');
      | for len=2:length(dtrid_b)
      | Splitname=regexp(Event_Id,'_','all');
      | New_EventId=insertBefore(Event_Id,Splitname(end),num2str(len));
      | eval([char(New_EventId) '= 0;']);
      | set_param(dtrid_b{len},'Value',char(New_EventId));
      | end
      | 
      | % ctrlval_b1 = find_system(gcb,'LookUnderMasks','all','FollowLinks','on','Name','Ctrlval_block1');
      | % ctrlval_b2 = find_system(gcb,'LookUnderMasks','all','FollowLinks','on','Name','Ctrlval_block2');
      | % ctrlval_b3 = find_system(gcb,'LookUnderMasks','all','FollowLinks','on','Name','Ctrlval_block3');
      | % ctrlval_b4 = find_system(gcb,'LookUnderMasks','all','FollowLinks','on','Name','Ctrlval_block4');
      | % ctrlval_b5 = find_system(gcb,'LookUnderMasks','all','FollowLinks','on','Name','Ctrlval_block5');
      | % ctrlval_b6 = find_system(gcb,'LookUnderMasks','all','FollowLinks','on','Name','Ctrlval_block6');
      | % ctrlval_b7 = find_system(gcb,'LookUnderMasks','all','FollowLinks','on','Name','Ctrlval_block7');
      | % ctrlval_b8 = find_system(gcb,'LookUnderMasks','all','FollowLinks','on','Name','Ctrlval_block8');
      | 
      | resol_b3 = find_system(gcb,'LookUnderMasks','all','FollowLinks','on','Name','Resolution_block1');
      | resol_b4 = find_system(gcb,'LookUnderMasks','all','FollowLinks','on','Name','Resolution_block2');
      | resol_b5 = find_system(gcb,'LookUnderMasks','all','FollowLinks','on','Name','Resolution_block3');
      | resol_b6 = find_system(gcb,'LookUnderMasks','all','FollowLinks','on','Name','Resolution_block4');
      | resol_b7 = find_system(gcb,'LookUnderMasks','all','FollowLinks','on','Name','Resolution_block5');
      | resol_b8 = find_system(gcb,'LookUnderMasks','all','FollowLinks','on','Name','Resolution_block6');
      | resol_b9 = find_system(gcb,'LookUnderMasks','all','FollowLinks','on','Name','Resolution_block7');
      | resol_b10 = find_system(gcb,'LookUnderMasks','all','FollowLinks','on','Name','Resolution_block8');
      | resol_b11 = find_system(gcb,'LookUnderMasks','all','FollowLinks','on','Name','Resolution_block9');
      | resol_b12 = find_system(gcb,'LookUnderMasks','all','FollowLinks','on','Name','Resolution_block10');
      | resol_b13 = find_system(gcb,'LookUnderMasks','all','FollowLinks','on','Name','Resolution_block11');
      | resol_b14 = find_system(gcb,'LookUnderMasks','all','FollowLinks','on','Name','Resolution_block12');
      | resol_b15 = find_system(gcb,'LookUnderMasks','all','FollowLinks','on','Name','Resolution_block13');
      | resol_b16 = find_system(gcb,'LookUnderMasks','all','FollowLinks','on','Name','Resolution_block14');
      | resol_b17 = find_system(gcb,'LookUnderMasks','all','FollowLinks','on','Name','Resolution_block15');
      | resol_b18 = find_system(gcb,'LookUnderMasks','all','FollowLinks','on','Name','Resolution_block16');
      | resol_b19 = find_system(gcb,'LookUnderMasks','all','FollowLinks','on','Name','Resolution_block17');
      | resol_b20 = find_system(gcb,'LookUnderMasks','all','FollowLinks','on','Name','Resolution_block18');
      | resol_b21 = find_system(gcb,'LookUnderMasks','all','FollowLinks','on','Name','Resolution_block19');
      | resol_b22 = find_system(gcb,'LookUnderMasks','all','FollowLinks','on','Name','Resolution_block20');
      | resol_b23 = find_system(gcb,'LookUnderMasks','all','FollowLinks','on','Name','Resolution_block21');
      | resol_b24 = find_system(gcb,'LookUnderMasks','all','FollowLinks','on','Name','Resolution_block22');
      | resol_b25 = find_system(gcb,'LookUnderMasks','all','FollowLinks','on','Name','Resolution_block23');
      | resol_b26 = find_system(gcb,'LookUnderMasks','all','FollowLinks','on','Name','Resolution_block24');
      | 
      | limit_b1 = find_system(gcb,'LookUnderMasks','all','FollowLinks','on','Name','Limitter1');
      | limit_b2 = find_system(gcb,'LookUnderMasks','all','FollowLinks','on','Name','Limitter2');
      | limit_b3 = find_system(gcb,'LookUnderMasks','all','FollowLinks','on','Name','Limitter3');
      | limit_b4 = find_system(gcb,'LookUnderMasks','all','FollowLinks','on','Name','Limitter4');
      | limit_b5 = find_system(gcb,'LookUnderMasks','all','FollowLinks','on','Name','Limitter5');
      | limit_b6 = find_system(gcb,'LookUnderMasks','all','FollowLinks','on','Name','Limitter6');
      | limit_b7 = find_system(gcb,'LookUnderMasks','all','FollowLinks','on','Name','Limitter7');
      | limit_b8 = find_system(gcb,'LookUnderMasks','all','FollowLinks','on','Name','Limitter8');
      | limit_b9 = find_system(gcb,'LookUnderMasks','all','FollowLinks','on','Name','Limitter9');
      | limit_b10 = find_system(gcb,'LookUnderMasks','all','FollowLinks','on','Name','Limitter10');
      | limit_b11 = find_system(gcb,'LookUnderMasks','all','FollowLinks','on','Name','Limitter11');
      | limit_b12 = find_system(gcb,'LookUnderMasks','all','FollowLinks','on','Name','Limitter12');
      | limit_b13 = find_system(gcb,'LookUnderMasks','all','FollowLinks','on','Name','Limitter13');
      | limit_b14 = find_system(gcb,'LookUnderMasks','all','FollowLinks','on','Name','Limitter14');
      | limit_b15 = find_system(gcb,'LookUnderMasks','all','FollowLinks','on','Name','Limitter15');
      | limit_b16 = find_system(gcb,'LookUnderMasks','all','FollowLinks','on','Name','Limitter16');
      | limit_b17 = find_system(gcb,'LookUnderMasks','all','FollowLinks','on','Name','Limitter17');
      | limit_b18 = find_system(gcb,'LookUnderMasks','all','FollowLinks','on','Name','Limitter18');
      | limit_b19 = find_system(gcb,'LookUnderMasks','all','FollowLinks','on','Name','Limitter19');
      | limit_b20 = find_system(gcb,'LookUnderMasks','all','FollowLinks','on','Name','Limitter20');
      | limit_b21 = find_system(gcb,'LookUnderMasks','all','FollowLinks','on','Name','Limitter21');
      | limit_b22 = find_system(gcb,'LookUnderMasks','all','FollowLinks','on','Name','Limitter22');
      | limit_b23 = find_system(gcb,'LookUnderMasks','all','FollowLinks','on','Name','Limitter23');
      | limit_b24 = find_system(gcb,'LookUnderMasks','all','FollowLinks','on','Name','Limitter24');
      | 
      | 
      | % for n = 1:length(ctrlval_b1)
      | %     set_param([ctrlval_b1{n}],'Value',[char(Ctrlval) '_1']);
      | %     set_param([ctrlval_b2{n}],'Value',[char(Ctrlval) '_2']);
      | %     set_param([ctrlval_b3{n}],'Value',[char(Ctrlval) '_3']);
      | %     set_param([ctrlval_b4{n}],'Value',[char(Ctrlval) '_4']);
      | %     set_param([ctrlval_b5{n}],'Value',[char(Ctrlval) '_5']);
      | %     set_param([ctrlval_b6{n}],'Value',[char(Ctrlval) '_6']);
      | %     set_param([ctrlval_b7{n}],'Value',[char(Ctrlval) '_7']);
      | %     set_param([ctrlval_b8{n}],'Value',[char(Ctrlval) '_8']);
      | % end
      | 
      | set_param([resol_b1{:}],'Value',resol);
      | set_param([resol_b2{:}],'Value',resol);
      | set_param([resol_b3{:}],'Value',resol);
      | set_param([resol_b4{:}],'Value',resol);
      | set_param([resol_b5{:}],'Value',resol);
      | set_param([resol_b6{:}],'Value',resol);
      | set_param([resol_b7{:}],'Value',resol);
      | set_param([resol_b8{:}],'Value',resol);
      | set_param([resol_b9{:}],'Value',resol);
      | set_param([resol_b10{:}],'Value',resol);
      | set_param([resol_b11{:}],'Value',resol);
      | set_param([resol_b12{:}],'Value',resol);
      | set_param([resol_b13{:}],'Value',resol);
      | set_param([resol_b14{:}],'Value',resol);
      | set_param([resol_b15{:}],'Value',resol);
      | set_param([resol_b16{:}],'Value',resol);
      | set_param([resol_b17{:}],'Value',resol);
      | set_param([resol_b18{:}],'Value',resol);
      | set_param([resol_b19{:}],'Value',resol);
      | set_param([resol_b20{:}],'Value',resol);
      | set_param([resol_b21{:}],'Value',resol);
      | set_param([resol_b22{:}],'Value',resol);
      | set_param([resol_b23{:}],'Value',resol);
      | set_param([resol_b24{:}],'Value',resol);
      | set_param([resol_b25{:}],'Value',resol);
      | set_param([resol_b26{:}],'Value',resol);
      |  
      | set_param([limit_b1{:}],'UpperLimit',ulim);
      | set_param([limit_b2{:}],'UpperLimit',ulim);
      | set_param([limit_b3{:}],'UpperLimit',ulim);
      | set_param([limit_b4{:}],'UpperLimit',ulim);
      | set_param([limit_b5{:}],'UpperLimit',ulim);
      | set_param([limit_b6{:}],'UpperLimit',ulim);        
      | set_param([limit_b7{:}],'UpperLimit',ulim);
      | set_param([limit_b8{:}],'UpperLimit',ulim);
      | set_param([limit_b9{:}],'UpperLimit',ulim);
      | set_param([limit_b10{:}],'UpperLimit',ulim);
      | set_param([limit_b11{:}],'UpperLimit',ulim);
      | set_param([limit_b12{:}],'UpperLimit',ulim);
      | set_param([limit_b13{:}],'UpperLimit',ulim);
      | set_param([limit_b14{:}],'UpperLimit',ulim);
      | set_param([limit_b15{:}],'UpperLimit',ulim);
      | set_param([limit_b16{:}],'UpperLimit',ulim);
      | set_param([limit_b17{:}],'UpperLimit',ulim);
      | set_param([limit_b18{:}],'UpperLimit',ulim);
      | set_param([limit_b19{:}],'UpperLimit',ulim);
      | set_param([limit_b20{:}],'UpperLimit',ulim);
      | set_param([limit_b21{:}],'UpperLimit',ulim);
      | set_param([limit_b22{:}],'UpperLimit',ulim);
      | set_param([limit_b23{:}],'UpperLimit',ulim);
      | set_param([limit_b24{:}],'UpperLimit',ulim);
      |  
      | set_param([limit_b1{:}],'LowerLimit',dlim);
      | set_param([limit_b2{:}],'LowerLimit',dlim);
      | set_param([limit_b3{:}],'LowerLimit',dlim);
      | set_param([limit_b4{:}],'LowerLimit',dlim);
      | set_param([limit_b5{:}],'LowerLimit',dlim);
      | set_param([limit_b6{:}],'LowerLimit',dlim);
      | set_param([limit_b7{:}],'LowerLimit',dlim);
      | set_param([limit_b8{:}],'LowerLimit',dlim);
      | set_param([limit_b9{:}],'LowerLimit',dlim);
      | set_param([limit_b10{:}],'LowerLimit',dlim);
      | set_param([limit_b11{:}],'LowerLimit',dlim);
      | set_param([limit_b12{:}],'LowerLimit',dlim);
      | set_param([limit_b13{:}],'LowerLimit',dlim);
      | set_param([limit_b14{:}],'LowerLimit',dlim);
      | set_param([limit_b15{:}],'LowerLimit',dlim);
      | set_param([limit_b16{:}],'LowerLimit',dlim);
      | set_param([limit_b17{:}],'LowerLimit',dlim);
      | set_param([limit_b18{:}],'LowerLimit',dlim);
      | set_param([limit_b19{:}],'LowerLimit',dlim);
      | set_param([limit_b20{:}],'LowerLimit',dlim);
      | set_param([limit_b21{:}],'LowerLimit',dlim);
      | set_param([limit_b22{:}],'LowerLimit',dlim);
      | set_param([limit_b23{:}],'LowerLimit',dlim);
      | set_param([limit_b24{:}],'LowerLimit',dlim);
      settings: AttributesFormatString=%<MaskType>\nConversion Type : = %<conv_type>\nEventId = %<EventId>\nreslution = %<resol>\nlowerlimit = %<dlim>\nupperlimit = %<ulim>
      mask TypeOptions conv_type: 0x01 | 0x02 | 0x03 | 0x04 | 0x05 | 0x06 | 0x07 | 0x08 | 0x09 | 0x0A | 0x0B | 0x0C | 0x0D | 0x0E | 0x0F | 0x10 | 0x11 | 0x12 | 0x13 | 0x14 | 0x15 | 0x16 | 0x17 | 0x18 | 0x19 | 0x1A | 0x1B | 0x1C | 0x1D | 0x1E | 0x1F | 0x20 | 0x21 | 0x22 | 0x23 | 0x24 | 0x25 | 0x26 | 0x27 | 0x28 | 0x29 | 0x2A | 0x2B | 0x2C | 0x2D | 0x2E | 0x2F | 0x30 | 0x31 | 0x32 | 0x33 | 0x34 | 0x35 | 0x36 | 0x37 | 0x38 | 0x39 | 0x3A | 0x3B | 0x3C | 0x3D | 0x3E | 0x3F | 0x40 | 0x41 | 0x42 | 0x43 | 0x44 | 0x81 | 0x82 | 0x83 | 0x84 | 0x85 | 0x86 | 0x87 | 0x8A | 0x8B | 0x8C | 0x8D | 0x8E | 0x8F | 0x90 | 0x91 | 0x92 | 0x96 | 0x97 | 0x98 | 0x99 | 0x9C | 0x9D | 0xA8 | 0xA9 | 0xAD | 0xAE | 0xAF | 0xB0 | 0xB1 | 0xFA | 0xFB | 0xFC | 0xFD | 0xFE
      mask Display:
      | port_label('input',1,'set_flag');
      | port_label('input',2,'testresult');
      | port_label('input',3,'lowerlimit');
      | port_label('input',4,'upperlimit');
      | port_label('input',5,'ctrl_flag');
      | 
      | dgn_mask = [char(EventId) '\n Conversion : ' conv_type];
      | 
      | disp(dgn_mask);
      | 
      | plot([5,5,5])
      | plot([6,6,6])
  AEMS_DEM_SET_DTR_8DU : Subsystem  Tag=[LIB]  mask(AEMS_DEM_SET_DTR_8DU){conv_type=0x24, EventId=Dem_DtrId_XXX, resol=1, dlim=0, ulim=1}
      mask prompts: conv_type "Conversion Type :"; resol "resolution"; dlim "lowerlimit"; ulim "upperlimit"
      mask init:
      | % eval([char(EventId) '_1 = 0;']);
      | % eval([char(EventId) '_2 = 0;']);
      | % eval([char(EventId) '_3 = 0;']);
      | % eval([char(EventId) '_4 = 0;']);
      | % eval([char(EventId) '_5 = 0;']);
      | % eval([char(EventId) '_6 = 0;']);
      | % eval([char(EventId) '_7 = 0;']);
      | % eval([char(EventId) '_8 = 0;']);
      | % eval([char(Ctrlval) '_1 = 0;']);
      | % eval([char(Ctrlval) '_2 = 0;']);
      | % eval([char(Ctrlval) '_3 = 0;']);
      | % eval([char(Ctrlval) '_4 = 0;']);
      | % eval([char(Ctrlval) '_5 = 0;']);
      | % eval([char(Ctrlval) '_6 = 0;']);
      | % eval([char(Ctrlval) '_7 = 0;']);
      | % eval([char(Ctrlval) '_8 = 0;']);
      | eval(['DEM_DTR_CTL_NORMAL = 0;']);
      | eval(['DEM_DTR_CTL_INVISIBLE = 4;']);
      | 
      | Event_Id=get_param(gcb,'EventId');
      | 
      | dtrid_b1 = find_system(gcb,'LookUnderMasks','all','FollowLinks','on','Name','DTRId_block1');
      | eval([char(Event_Id) '= 0;']);
      | set_param(dtrid_b1{:},'Value',char(Event_Id));
      | 
      | dtrid_b = find_system(gcb,'LookUnderMasks','all','FollowLinks','on','regexp','on','Name','^DTRId_block');
      | for len=2:length(dtrid_b)
      | Splitname=regexp(Event_Id,'_','all');
      | New_EventId=insertBefore(Event_Id,Splitname(end),num2str(len));
      | eval([char(New_EventId) '= 0;']);
      | set_param(dtrid_b{len},'Value',char(New_EventId));
      | end
      | 
      | % dtrid_b1 = find_system(gcb,'LookUnderMasks','all','FollowLinks','on','Name','DTRId_block1');
      | % dtrid_b2 = find_system(gcb,'LookUnderMasks','all','FollowLinks','on','Name','DTRId_block2');
      | % dtrid_b3 = find_system(gcb,'LookUnderMasks','all','FollowLinks','on','Name','DTRId_block3');
      | % dtrid_b4 = find_system(gcb,'LookUnderMasks','all','FollowLinks','on','Name','DTRId_block4');
      | % dtrid_b5 = find_system(gcb,'LookUnderMasks','all','FollowLinks','on','Name','DTRId_block5');
      | % dtrid_b6 = find_system(gcb,'LookUnderMasks','all','FollowLinks','on','Name','DTRId_block6');
      | % dtrid_b7 = find_system(gcb,'LookUnderMasks','all','FollowLinks','on','Name','DTRId_block7');
      | % dtrid_b8 = find_system(gcb,'LookUnderMasks','all','FollowLinks','on','Name','DTRId_block8');
      | 
      | % ctrlval_b1 = find_system(gcb,'LookUnderMasks','all','FollowLinks','on','Name','Ctrlval_block1');
      | % ctrlval_b2 = find_system(gcb,'LookUnderMasks','all','FollowLinks','on','Name','Ctrlval_block2');
      | % ctrlval_b3 = find_system(gcb,'LookUnderMasks','all','FollowLinks','on','Name','Ctrlval_block3');
      | % ctrlval_b4 = find_system(gcb,'LookUnderMasks','all','FollowLinks','on','Name','Ctrlval_block4');
      | % ctrlval_b5 = find_system(gcb,'LookUnderMasks','all','FollowLinks','on','Name','Ctrlval_block5');
      | % ctrlval_b6 = find_system(gcb,'LookUnderMasks','all','FollowLinks','on','Name','Ctrlval_block6');
      | % ctrlval_b7 = find_system(gcb,'LookUnderMasks','all','FollowLinks','on','Name','Ctrlval_block7');
      | % ctrlval_b8 = find_system(gcb,'LookUnderMasks','all','FollowLinks','on','Name','Ctrlval_block8');
      | 
      | %offsetblock is not been set. Please add if requested.
      | limit_b1 = find_system(gcb,'LookUnderMasks','all','FollowLinks','on','Name','Limitter1');
      | limit_b2 = find_system(gcb,'LookUnderMasks','all','FollowLinks','on','Name','Limitter2');
      | limit_b3 = find_system(gcb,'LookUnderMasks','all','FollowLinks','on','Name','Limitter3');
      | limit_b4 = find_system(gcb,'LookUnderMasks','all','FollowLinks','on','Name','Limitter4');
      | limit_b5 = find_system(gcb,'LookUnderMasks','all','FollowLinks','on','Name','Limitter5');
      | limit_b6 = find_system(gcb,'LookUnderMasks','all','FollowLinks','on','Name','Limitter6');
      | limit_b7 = find_system(gcb,'LookUnderMasks','all','FollowLinks','on','Name','Limitter7');
      | limit_b8 = find_system(gcb,'LookUnderMasks','all','FollowLinks','on','Name','Limitter8');
      | limit_b9 = find_system(gcb,'LookUnderMasks','all','FollowLinks','on','Name','Limitter9');
      | limit_b10 = find_system(gcb,'LookUnderMasks','all','FollowLinks','on','Name','Limitter10');
      | limit_b11 = find_system(gcb,'LookUnderMasks','all','FollowLinks','on','Name','Limitter11');
      | limit_b12 = find_system(gcb,'LookUnderMasks','all','FollowLinks','on','Name','Limitter12');
      | limit_b13 = find_system(gcb,'LookUnderMasks','all','FollowLinks','on','Name','Limitter13');
      | limit_b14 = find_system(gcb,'LookUnderMasks','all','FollowLinks','on','Name','Limitter14');
      | limit_b15 = find_system(gcb,'LookUnderMasks','all','FollowLinks','on','Name','Limitter15');
      | limit_b16 = find_system(gcb,'LookUnderMasks','all','FollowLinks','on','Name','Limitter16');
      | limit_b17 = find_system(gcb,'LookUnderMasks','all','FollowLinks','on','Name','Limitter17');
      | limit_b18 = find_system(gcb,'LookUnderMasks','all','FollowLinks','on','Name','Limitter18');
      | limit_b19 = find_system(gcb,'LookUnderMasks','all','FollowLinks','on','Name','Limitter19');
      | limit_b20 = find_system(gcb,'LookUnderMasks','all','FollowLinks','on','Name','Limitter20');
      | limit_b21 = find_system(gcb,'LookUnderMasks','all','FollowLinks','on','Name','Limitter21');
      | limit_b22 = find_system(gcb,'LookUnderMasks','all','FollowLinks','on','Name','Limitter22');
      | limit_b23 = find_system(gcb,'LookUnderMasks','all','FollowLinks','on','Name','Limitter23');
      | limit_b24 = find_system(gcb,'LookUnderMasks','all','FollowLinks','on','Name','Limitter24');
      | 
      | % for n = 1:length(dtrid_b1)
      | %     set_param([dtrid_b1{n}],'Value',[char(EventId) '_1']);
      | %     set_param([dtrid_b2{n}],'Value',[char(EventId) '_2']);
      | %     set_param([dtrid_b3{n}],'Value',[char(EventId) '_3']);
      | %     set_param([dtrid_b4{n}],'Value',[char(EventId) '_4']);
      | %     set_param([dtrid_b5{n}],'Value',[char(EventId) '_5']);
      | %     set_param([dtrid_b6{n}],'Value',[char(EventId) '_6']);
      | %     set_param([dtrid_b7{n}],'Value',[char(EventId) '_7']);
      | %     set_param([dtrid_b8{n}],'Value',[char(EventId) '_8']); 
      | % end
      | 
      | % for n = 1:length(ctrlval_b1)
      | %     set_param([ctrlval_b1{n}],'Value',[char(Ctrlval) '_1']);
      | %     set_param([ctrlval_b2{n}],'Value',[char(Ctrlval) '_2']);
      | %     set_param([ctrlval_b3{n}],'Value',[char(Ctrlval) '_3']);
      | %     set_param([ctrlval_b4{n}],'Value',[char(Ctrlval) '_4']);
      | %     set_param([ctrlval_b5{n}],'Value',[char(Ctrlval) '_5']);
      | %     set_param([ctrlval_b6{n}],'Value',[char(Ctrlval) '_6']);
      | %     set_param([ctrlval_b7{n}],'Value',[char(Ctrlval) '_7']);
      | %     set_param([ctrlval_b8{n}],'Value',[char(Ctrlval) '_8']);
      | % end
      | 
      | set_param([limit_b1{:}],'UpperLimit',ulim);
      | set_param([limit_b2{:}],'UpperLimit',ulim);
      | set_param([limit_b3{:}],'UpperLimit',ulim);
      | set_param([limit_b4{:}],'UpperLimit',ulim);
      | set_param([limit_b5{:}],'UpperLimit',ulim);
      | set_param([limit_b6{:}],'UpperLimit',ulim);        
      | set_param([limit_b7{:}],'UpperLimit',ulim);
      | set_param([limit_b8{:}],'UpperLimit',ulim);
      | set_param([limit_b9{:}],'UpperLimit',ulim);
      | set_param([limit_b10{:}],'UpperLimit',ulim);
      | set_param([limit_b11{:}],'UpperLimit',ulim);
      | set_param([limit_b12{:}],'UpperLimit',ulim);
      | set_param([limit_b13{:}],'UpperLimit',ulim);
      | set_param([limit_b14{:}],'UpperLimit',ulim);
      | set_param([limit_b15{:}],'UpperLimit',ulim);
      | set_param([limit_b16{:}],'UpperLimit',ulim);
      | set_param([limit_b17{:}],'UpperLimit',ulim);
      | set_param([limit_b18{:}],'UpperLimit',ulim);
      | set_param([limit_b19{:}],'UpperLimit',ulim);
      | set_param([limit_b20{:}],'UpperLimit',ulim);
      | set_param([limit_b21{:}],'UpperLimit',ulim);
      | set_param([limit_b22{:}],'UpperLimit',ulim);
      | set_param([limit_b23{:}],'UpperLimit',ulim);
      | set_param([limit_b24{:}],'UpperLimit',ulim);
      |  
      | set_param([limit_b1{:}],'LowerLimit',dlim);
      | set_param([limit_b2{:}],'LowerLimit',dlim);
      | set_param([limit_b3{:}],'LowerLimit',dlim);
      | set_param([limit_b4{:}],'LowerLimit',dlim);
      | set_param([limit_b5{:}],'LowerLimit',dlim);
      | set_param([limit_b6{:}],'LowerLimit',dlim);
      | set_param([limit_b7{:}],'LowerLimit',dlim);
      | set_param([limit_b8{:}],'LowerLimit',dlim);
      | set_param([limit_b9{:}],'LowerLimit',dlim);
      | set_param([limit_b10{:}],'LowerLimit',dlim);
      | set_param([limit_b11{:}],'LowerLimit',dlim);
      | set_param([limit_b12{:}],'LowerLimit',dlim);
      | set_param([limit_b13{:}],'LowerLimit',dlim);
      | set_param([limit_b14{:}],'LowerLimit',dlim);
      | set_param([limit_b15{:}],'LowerLimit',dlim);
      | set_param([limit_b16{:}],'LowerLimit',dlim);
      | set_param([limit_b17{:}],'LowerLimit',dlim);
      | set_param([limit_b18{:}],'LowerLimit',dlim);
      | set_param([limit_b19{:}],'LowerLimit',dlim);
      | set_param([limit_b20{:}],'LowerLimit',dlim);
      | set_param([limit_b21{:}],'LowerLimit',dlim);
      | set_param([limit_b22{:}],'LowerLimit',dlim);
      | set_param([limit_b23{:}],'LowerLimit',dlim);
      | set_param([limit_b24{:}],'LowerLimit',dlim);
      settings: AttributesFormatString=%<MaskType>\nConversion Type : = %<conv_type>\nEventId = %<EventId>\nresolution = %<resol>\nlowerlimit = %<dlim>\nupperlimit = %<ulim>
      mask TypeOptions conv_type: 0x01 | 0x02 | 0x03 | 0x04 | 0x05 | 0x06 | 0x07 | 0x08 | 0x09 | 0x0A | 0x0B | 0x0C | 0x0D | 0x0E | 0x0F | 0x10 | 0x11 | 0x12 | 0x13 | 0x14 | 0x15 | 0x16 | 0x17 | 0x18 | 0x19 | 0x1A | 0x1B | 0x1C | 0x1D | 0x1E | 0x1F | 0x20 | 0x21 | 0x22 | 0x23 | 0x24 | 0x25 | 0x26 | 0x27 | 0x28 | 0x29 | 0x2A | 0x2B | 0x2C | 0x2D | 0x2E | 0x2F | 0x30 | 0x31 | 0x32 | 0x33 | 0x34 | 0x35 | 0x36 | 0x37 | 0x38 | 0x39 | 0x3A | 0x3B | 0x3C | 0x3D | 0x3E | 0x3F | 0x40 | 0x41 | 0x42 | 0x43 | 0x44 | 0x81 | 0x82 | 0x83 | 0x84 | 0x85 | 0x86 | 0x87 | 0x8A | 0x8B | 0x8C | 0x8D | 0x8E | 0x8F | 0x90 | 0x91 | 0x92 | 0x96 | 0x97 | 0x98 | 0x99 | 0x9C | 0x9D | 0xA8 | 0xA9 | 0xAD | 0xAE | 0xAF | 0xB0 | 0xB1 | 0xFA | 0xFB | 0xFC | 0xFD | 0xFE
      mask Display:
      | port_label('input',1,'set_flag');
      | port_label('input',2,'testresult');
      | port_label('input',3,'lowerlimit');
      | port_label('input',4,'upperlimit');
      | port_label('input',5,'ctrl_flag');
      | 
      | dgn_mask = [char(EventId) '\n Conversion : ' conv_type];
      | 
      | disp(dgn_mask);
      | 
      | plot([5,5,5])
      | plot([6,6,6])
  AEMS_DEM_SET_DTR_9DU : Subsystem  Tag=[LIB]  mask(AEMS_DEM_SET_DTR_9DU){conv_type=0x24, EventId=Dem_DtrId_XXX, resol=1, dlim=0, ulim=1}
      mask prompts: conv_type "Conversion Type :"; resol "resolution"; dlim "lowerlimit"; ulim "upperlimit"
      mask init:
      | % eval([char(EventId) '_0 = 0;']);
      | % eval([char(EventId) '_1 = 0;']);
      | % eval([char(EventId) '_2 = 0;']);
      | % eval([char(EventId) '_3 = 0;']);
      | % eval([char(EventId) '_4 = 0;']);
      | % eval([char(EventId) '_5 = 0;']);
      | % eval([char(EventId) '_6 = 0;']);
      | % eval([char(EventId) '_7 = 0;']);
      | % eval([char(EventId) '_8 = 0;']);
      | % eval([char(Ctrlval) '_1 = 0;']);
      | % eval([char(Ctrlval) '_2 = 0;']);
      | % eval([char(Ctrlval) '_3 = 0;']);
      | % eval([char(Ctrlval) '_4 = 0;']);
      | % eval([char(Ctrlval) '_5 = 0;']);
      | % eval([char(Ctrlval) '_6 = 0;']);
      | % eval([char(Ctrlval) '_7 = 0;']);
      | % eval([char(Ctrlval) '_8 = 0;']);
      | eval(['DEM_DTR_CTL_NORMAL = 0;']);
      | eval(['DEM_DTR_CTL_INVISIBLE = 4;']);
      | 
      | Event_Id=get_param(gcb,'EventId');
      | 
      | dtrid_b0 = find_system(gcb,'LookUnderMasks','all','FollowLinks','on','Name','DTRId_block0');
      | eval([char(Event_Id) '= 0;']);
      | set_param(dtrid_b0{:},'Value',char(Event_Id));
      | 
      | dtrid_b = find_system(gcb,'LookUnderMasks','all','FollowLinks','on','regexp','on','Name','^DTRId_block');
      | for len=2:length(dtrid_b)
      | Splitname=regexp(Event_Id,'_','all');
      | New_EventId=insertBefore(Event_Id,Splitname(end),num2str(len));
      | eval([char(New_EventId) '= 0;']);
      | set_param(dtrid_b{len},'Value',char(New_EventId));
      | end
      | 
      | 
      | % dtrid_b0 = find_system(gcb,'LookUnderMasks','all','FollowLinks','on','Name','DTRId_block0');
      | % dtrid_b1 = find_system(gcb,'LookUnderMasks','all','FollowLinks','on','Name','DTRId_block1');
      | % dtrid_b2 = find_system(gcb,'LookUnderMasks','all','FollowLinks','on','Name','DTRId_block2');
      | % dtrid_b3 = find_system(gcb,'LookUnderMasks','all','FollowLinks','on','Name','DTRId_block3');
      | % dtrid_b4 = find_system(gcb,'LookUnderMasks','all','FollowLinks','on','Name','DTRId_block4');
      | % dtrid_b5 = find_system(gcb,'LookUnderMasks','all','FollowLinks','on','Name','DTRId_block5');
      | % dtrid_b6 = find_system(gcb,'LookUnderMasks','all','FollowLinks','on','Name','DTRId_block6');
      | % dtrid_b7 = find_system(gcb,'LookUnderMasks','all','FollowLinks','on','Name','DTRId_block7');
      | % dtrid_b8 = find_system(gcb,'LookUnderMasks','all','FollowLinks','on','Name','DTRId_block8');
      | 
      | % ctrlval_b1 = find_system(gcb,'LookUnderMasks','all','FollowLinks','on','Name','Ctrlval_block1');
      | % ctrlval_b2 = find_system(gcb,'LookUnderMasks','all','FollowLinks','on','Name','Ctrlval_block2');
      | % ctrlval_b3 = find_system(gcb,'LookUnderMasks','all','FollowLinks','on','Name','Ctrlval_block3');
      | % ctrlval_b4 = find_system(gcb,'LookUnderMasks','all','FollowLinks','on','Name','Ctrlval_block4');
      | % ctrlval_b5 = find_system(gcb,'LookUnderMasks','all','FollowLinks','on','Name','Ctrlval_block5');
      | % ctrlval_b6 = find_system(gcb,'LookUnderMasks','all','FollowLinks','on','Name','Ctrlval_block6');
      | % ctrlval_b7 = find_system(gcb,'LookUnderMasks','all','FollowLinks','on','Name','Ctrlval_block7');
      | % ctrlval_b8 = find_system(gcb,'LookUnderMasks','all','FollowLinks','on','Name','Ctrlval_block8');
      | 
      | %offsetblock is not been set. Please add if requested.
      | limit_b1 = find_system(gcb,'LookUnderMasks','all','FollowLinks','on','Name','Limitter1');
      | limit_b2 = find_system(gcb,'LookUnderMasks','all','FollowLinks','on','Name','Limitter2');
      | limit_b3 = find_system(gcb,'LookUnderMasks','all','FollowLinks','on','Name','Limitter3');
      | limit_b4 = find_system(gcb,'LookUnderMasks','all','FollowLinks','on','Name','Limitter4');
      | limit_b5 = find_system(gcb,'LookUnderMasks','all','FollowLinks','on','Name','Limitter5');
      | limit_b6 = find_system(gcb,'LookUnderMasks','all','FollowLinks','on','Name','Limitter6');
      | limit_b7 = find_system(gcb,'LookUnderMasks','all','FollowLinks','on','Name','Limitter7');
      | limit_b8 = find_system(gcb,'LookUnderMasks','all','FollowLinks','on','Name','Limitter8');
      | limit_b9 = find_system(gcb,'LookUnderMasks','all','FollowLinks','on','Name','Limitter9');
      | limit_b10 = find_system(gcb,'LookUnderMasks','all','FollowLinks','on','Name','Limitter10');
      | limit_b11 = find_system(gcb,'LookUnderMasks','all','FollowLinks','on','Name','Limitter11');
      | limit_b12 = find_system(gcb,'LookUnderMasks','all','FollowLinks','on','Name','Limitter12');
      | limit_b13 = find_system(gcb,'LookUnderMasks','all','FollowLinks','on','Name','Limitter13');
      | limit_b14 = find_system(gcb,'LookUnderMasks','all','FollowLinks','on','Name','Limitter14');
      | limit_b15 = find_system(gcb,'LookUnderMasks','all','FollowLinks','on','Name','Limitter15');
      | limit_b16 = find_system(gcb,'LookUnderMasks','all','FollowLinks','on','Name','Limitter16');
      | limit_b17 = find_system(gcb,'LookUnderMasks','all','FollowLinks','on','Name','Limitter17');
      | limit_b18 = find_system(gcb,'LookUnderMasks','all','FollowLinks','on','Name','Limitter18');
      | limit_b19 = find_system(gcb,'LookUnderMasks','all','FollowLinks','on','Name','Limitter19');
      | limit_b20 = find_system(gcb,'LookUnderMasks','all','FollowLinks','on','Name','Limitter20');
      | limit_b21 = find_system(gcb,'LookUnderMasks','all','FollowLinks','on','Name','Limitter21');
      | limit_b22 = find_system(gcb,'LookUnderMasks','all','FollowLinks','on','Name','Limitter22');
      | limit_b23 = find_system(gcb,'LookUnderMasks','all','FollowLinks','on','Name','Limitter23');
      | limit_b24 = find_system(gcb,'LookUnderMasks','all','FollowLinks','on','Name','Limitter24');
      | limit_b25 = find_system(gcb,'LookUnderMasks','all','FollowLinks','on','Name','Limitter25');
      | limit_b26 = find_system(gcb,'LookUnderMasks','all','FollowLinks','on','Name','Limitter26');
      | limit_b27 = find_system(gcb,'LookUnderMasks','all','FollowLinks','on','Name','Limitter27');
      | 
      | 
      | % for n = 1:length(dtrid_b1)
      | %     set_param([dtrid_b0{n}],'Value',[char(EventId) '_0']);
      | %     set_param([dtrid_b1{n}],'Value',[char(EventId) '_1']);
      | %     set_param([dtrid_b2{n}],'Value',[char(EventId) '_2']);
      | %     set_param([dtrid_b3{n}],'Value',[char(EventId) '_3']);
      | %     set_param([dtrid_b4{n}],'Value',[char(EventId) '_4']);
      | %     set_param([dtrid_b5{n}],'Value',[char(EventId) '_5']);
      | %     set_param([dtrid_b6{n}],'Value',[char(EventId) '_6']);
      | %     set_param([dtrid_b7{n}],'Value',[char(EventId) '_7']);
      | %     set_param([dtrid_b8{n}],'Value',[char(EventId) '_8']); 
      | % end
      | 
      | % for n = 1:length(ctrlval_b1)
      | %     set_param([ctrlval_b1{n}],'Value',[char(Ctrlval) '_1']);
      | %     set_param([ctrlval_b2{n}],'Value',[char(Ctrlval) '_2']);
      | %     set_param([ctrlval_b3{n}],'Value',[char(Ctrlval) '_3']);
      | %     set_param([ctrlval_b4{n}],'Value',[char(Ctrlval) '_4']);
      | %     set_param([ctrlval_b5{n}],'Value',[char(Ctrlval) '_5']);
      | %     set_param([ctrlval_b6{n}],'Value',[char(Ctrlval) '_6']);
      | %     set_param([ctrlval_b7{n}],'Value',[char(Ctrlval) '_7']);
      | %     set_param([ctrlval_b8{n}],'Value',[char(Ctrlval) '_8']);
      | % end
      | 
      | set_param([limit_b1{:}],'UpperLimit',ulim);
      | set_param([limit_b2{:}],'UpperLimit',ulim);
      | set_param([limit_b3{:}],'UpperLimit',ulim);
      | set_param([limit_b4{:}],'UpperLimit',ulim);
      | set_param([limit_b5{:}],'UpperLimit',ulim);
      | set_param([limit_b6{:}],'UpperLimit',ulim);        
      | set_param([limit_b7{:}],'UpperLimit',ulim);
      | set_param([limit_b8{:}],'UpperLimit',ulim);
      | set_param([limit_b9{:}],'UpperLimit',ulim);
      | set_param([limit_b10{:}],'UpperLimit',ulim);
      | set_param([limit_b11{:}],'UpperLimit',ulim);
      | set_param([limit_b12{:}],'UpperLimit',ulim);
      | set_param([limit_b13{:}],'UpperLimit',ulim);
      | set_param([limit_b14{:}],'UpperLimit',ulim);
      | set_param([limit_b15{:}],'UpperLimit',ulim);
      | set_param([limit_b16{:}],'UpperLimit',ulim);
      | set_param([limit_b17{:}],'UpperLimit',ulim);
      | set_param([limit_b18{:}],'UpperLimit',ulim);
      | set_param([limit_b19{:}],'UpperLimit',ulim);
      | set_param([limit_b20{:}],'UpperLimit',ulim);
      | set_param([limit_b21{:}],'UpperLimit',ulim);
      | set_param([limit_b22{:}],'UpperLimit',ulim);
      | set_param([limit_b23{:}],'UpperLimit',ulim);
      | set_param([limit_b24{:}],'UpperLimit',ulim);
      | set_param([limit_b25{:}],'UpperLimit',ulim);
      | set_param([limit_b26{:}],'UpperLimit',ulim);
      | set_param([limit_b27{:}],'UpperLimit',ulim);
      |  
      | set_param([limit_b1{:}],'LowerLimit',dlim);
      | set_param([limit_b2{:}],'LowerLimit',dlim);
      | set_param([limit_b3{:}],'LowerLimit',dlim);
      | set_param([limit_b4{:}],'LowerLimit',dlim);
      | set_param([limit_b5{:}],'LowerLimit',dlim);
      | set_param([limit_b6{:}],'LowerLimit',dlim);
      | set_param([limit_b7{:}],'LowerLimit',dlim);
      | set_param([limit_b8{:}],'LowerLimit',dlim);
      | set_param([limit_b9{:}],'LowerLimit',dlim);
      | set_param([limit_b10{:}],'LowerLimit',dlim);
      | set_param([limit_b11{:}],'LowerLimit',dlim);
      | set_param([limit_b12{:}],'LowerLimit',dlim);
      | set_param([limit_b13{:}],'LowerLimit',dlim);
      | set_param([limit_b14{:}],'LowerLimit',dlim);
      | set_param([limit_b15{:}],'LowerLimit',dlim);
      | set_param([limit_b16{:}],'LowerLimit',dlim);
      | set_param([limit_b17{:}],'LowerLimit',dlim);
      | set_param([limit_b18{:}],'LowerLimit',dlim);
      | set_param([limit_b19{:}],'LowerLimit',dlim);
      | set_param([limit_b20{:}],'LowerLimit',dlim);
      | set_param([limit_b21{:}],'LowerLimit',dlim);
      | set_param([limit_b22{:}],'LowerLimit',dlim);
      | set_param([limit_b23{:}],'LowerLimit',dlim);
      | set_param([limit_b24{:}],'LowerLimit',dlim);
      | set_param([limit_b25{:}],'LowerLimit',dlim);
      | set_param([limit_b26{:}],'LowerLimit',dlim);
      | set_param([limit_b27{:}],'LowerLimit',dlim);
      settings: AttributesFormatString=%<MaskType>\nConversion Type : = %<conv_type>\nEventId = %<EventId>\nresolution = %<resol>\nlowerlimit = %<dlim>\nupperlimit = %<ulim>
      mask TypeOptions conv_type: 0x01 | 0x02 | 0x03 | 0x04 | 0x05 | 0x06 | 0x07 | 0x08 | 0x09 | 0x0A | 0x0B | 0x0C | 0x0D | 0x0E | 0x0F | 0x10 | 0x11 | 0x12 | 0x13 | 0x14 | 0x15 | 0x16 | 0x17 | 0x18 | 0x19 | 0x1A | 0x1B | 0x1C | 0x1D | 0x1E | 0x1F | 0x20 | 0x21 | 0x22 | 0x23 | 0x24 | 0x25 | 0x26 | 0x27 | 0x28 | 0x29 | 0x2A | 0x2B | 0x2C | 0x2D | 0x2E | 0x2F | 0x30 | 0x31 | 0x32 | 0x33 | 0x34 | 0x35 | 0x36 | 0x37 | 0x38 | 0x39 | 0x3A | 0x3B | 0x3C | 0x3D | 0x3E | 0x3F | 0x40 | 0x41 | 0x42 | 0x43 | 0x44 | 0x81 | 0x82 | 0x83 | 0x84 | 0x85 | 0x86 | 0x87 | 0x8A | 0x8B | 0x8C | 0x8D | 0x8E | 0x8F | 0x90 | 0x91 | 0x92 | 0x96 | 0x97 | 0x98 | 0x99 | 0x9C | 0x9D | 0xA8 | 0xA9 | 0xAD | 0xAE | 0xAF | 0xB0 | 0xB1 | 0xFA | 0xFB | 0xFC | 0xFD | 0xFE
      mask Display:
      | port_label('input',1,'set_flag');
      | port_label('input',2,'testresult');
      | port_label('input',3,'lowerlimit');
      | port_label('input',4,'upperlimit');
      | port_label('input',5,'ctrl_flag');
      | 
      | dgn_mask = [char(EventId) '\n Conversion : ' conv_type];
      | 
      | disp(dgn_mask);
      | 
      | plot([5,5,5])
      | plot([6,6,6])
  AEMS_DEM_SET_ENBL_COND_1D : Subsystem  Tag=[LIB]  mask(AEMS_DEM_SET_ENBL_COND_1D){EnCondId=Dem_EnableConditionId_XXX}
      mask prompts: EnCondId "Enable Condition Id :"
      mask init:
      | eval([char(EnCondId) ' = 0;']);
      | 
      | encond_b1 = find_system(gcb,'LookUnderMasks','all','FollowLinks','on','Name','EnableConditionId_block');
      | 
      | set_param([encond_b1{:}],'Value',[char(EnCondId)]);
      settings: AttributesFormatString=%<MaskType>\nEnable Condition Id : = %<EnCondId>
      mask Display:
      | port_label('input',1,'conditionfulfilled');
      | 
      | dgn_mask = char(EnCondId);
      | 
      | disp(dgn_mask);
      | 
      | plot([5,5,5])
      | plot([6,6,6])
  AEMS_DEM_SET_ENBL_COND_2D : Subsystem  Tag=[LIB]  mask(AEMS_DEM_SET_ENBL_COND_2D){EnCondId=Dem_EnableConditionId_XXX}
      mask prompts: EnCondId "Enable Condition Id :"
      mask init:
      | This_Blk = gcb;
      | EnCond_Id=get_param(gcb,'EnCondId');
      | % eval([char(EnCondId) '_1 = 0;']);
      | % eval([char(EnCondId) '_2 = 0;']);
      | 
      | encond_b1 = find_system(This_Blk,'LookUnderMasks','all','FollowLinks','on','Name','EnableConditionId_block1');
      | eval([char(EnCond_Id) '= 0;']);
      | set_param(encond_b1{:},'Value',char(EnCond_Id));
      | 
      | encond_b2 = find_system(This_Blk,'LookUnderMasks','all','FollowLinks','on','Name','EnableConditionId_block2');
      | Splitname=regexp(EnCond_Id,'_','all');
      | EnCondId=insertBefore(EnCond_Id,Splitname(end),num2str(2));
      | eval([char(EnCondId) '= 0;']);
      | set_param(encond_b2{:},'Value',char(EnCondId));
      settings: AttributesFormatString=%<MaskType>\nEnable Condition Id : = %<EnCondId>
      mask Display:
      | port_label('input',1,'conditionfulfilled');
      | 
      | dgn_mask = char(EnCondId);
      | 
      | disp(dgn_mask);
      | 
      | plot([5,5,5])
      | plot([6,6,6])
  AEMS_DEM_SET_ENBL_COND_8D : Subsystem  Tag=[LIB]  mask(AEMS_DEM_SET_ENBL_COND_8D){EnCondId=Dem_EnableConditionId_XXX}
      mask prompts: EnCondId "Enable Condition Id :"
      mask init:
      | % eval([char(EnCondId) '_1 = 0;']);
      | % eval([char(EnCondId) '_2 = 0;']);
      | % eval([char(EnCondId) '_3 = 0;']);
      | % eval([char(EnCondId) '_4 = 0;']);
      | % eval([char(EnCondId) '_5 = 0;']);
      | % eval([char(EnCondId) '_6 = 0;']);
      | % eval([char(EnCondId) '_7 = 0;']);
      | % eval([char(EnCondId) '_8 = 0;']);
      | 
      | This_Blk = gcb;
      | EnCond_Id=get_param(gcb,'EnCondId');
      | 
      | encond_b1 = find_system(This_Blk,'LookUnderMasks','all','FollowLinks','on','Name','EnableConditionId_block1');
      | eval([char(EnCond_Id) '= 0;']);
      | set_param(encond_b1{:},'Value',char(EnCond_Id));
      | 
      | encond_b = find_system(This_Blk,'LookUnderMasks','all','FollowLinks','on','regexp','on','Name','^EnableConditionId_block');
      | for len=2:length(encond_b)
      | Splitname=regexp(EnCond_Id,'_','all');
      | EnCondId=insertBefore(EnCond_Id,Splitname(end),num2str(len));
      | eval([char(EnCondId) '= 0;']);
      | set_param(encond_b{len},'Value',char(EnCondId));
      | end
      settings: AttributesFormatString=%<MaskType>\nEnable Condition Id : = %<EnCondId>
      mask Display:
      | port_label('input',1,'conditionfulfilled');
      | 
      | dgn_mask = char(EnCondId);
      | 
      | disp(dgn_mask);
      | 
      | plot([5,5,5])
      | plot([6,6,6])
  AEMS_DEM_SET_EVENT_AVL_1D : Subsystem  Tag=[LIB]  mask(AEMS_DEM_SET_EVENT_AVL_1D){EventId=EventID, DiagROMFLAG=Diag_ROMFLAG}
      mask init:
      | eval([char(EventId) '= 0;'])%EventId is defined only in the library
      | 
      | %Specify constant block
      | eventid_b = find_system(gcb,'LookUnderMasks','all','FollowLinks','on','Name','EventId_block');
      | dgnsw_b = find_system(gcb,'LookUnderMasks','all','FollowLinks','on','Name','Diagnosis_SW');
      | % tsample_b = find_system(gcb,'LookUnderMasks','all','FollowLinks','on','Name','DEM_SET_EVENT_AVL_UD');
      | 
      | %Set value of constant
      | set_param([eventid_b{:}],'Value',char(EventId));
      | set_param([dgnsw_b{:}],'Value',char(DiagROMFLAG));
      | % set_param([tsample_b{:}],'SampleTime',char(sample_time));
      settings: AttributesFormatString=%<MaskType>\nEventId = %<EventId>\nDiagROMFLAG = %<DiagROMFLAG>
      mask Help:
      | eval('path_lib=fileparts(which(''AEMS_Standard_Library''));');
      | doc_path = [path_lib '\help\AEMS_DEM_SET_EVENT_AVL_1D.pdf'];
      | eval('open(doc_path)')
      mask Display:
      | dgn_mask = ['Event ID: ' char(EventId) '\n Diagnosis ROMFLAG: ' char(DiagROMFLAG)];
      | 
      | disp(dgn_mask);
      | plot([5,5,5])
      | plot([6,6,6])
  AEMS_DEM_SET_EVENT_AVL_2D : Subsystem  Tag=[LIB]  mask(AEMS_DEM_SET_EVENT_AVL_2D){EventId=Dem_EventId_XXX, DiagROMFLAG=mfXXX, sample_time=-1, immediate=Cnx_bnk_nr_conf}
      mask init:
      | % eval([char(EventId) '_1 = 0;'])%EventId is defined only in the library
      | % eval([char(EventId) '_2 = 0;'])%EventId is defined only in the library
      | 
      | %Specify constant block
      | dgnsw_b = find_system(gcb,'LookUnderMasks','all','FollowLinks','on','Name','Diagnosis_SW');
      | % eventid_b = find_system(gcb,'LookUnderMasks','all','FollowLinks','on','Name','EventId_block1');
      | % eventid_b1 = find_system(gcb,'LookUnderMasks','all','FollowLinks','on','Name','EventId_block2');
      | tsample_b = find_system(gcb,'LookUnderMasks','all','FollowLinks','on','Name','DEM_SET_EVENT_AVL_UD');
      | immt_b = find_system(gcb,'LookUnderMasks','all','FollowLinks','on','Name','index_parameter');
      | 
      | Event_Id=get_param(gcb,'EventId');
      | 
      | eventid_b = find_system(gcb,'LookUnderMasks','all','FollowLinks','on','regexp','on','Name','^EventId_block');
      | eventid_b1 = find_system(gcb,'LookUnderMasks','all','FollowLinks','on','Name','EventId_block1');
      | eval([char(Event_Id) '= 0;']);
      | set_param(eventid_b1{:},'Value',char(Event_Id));
      | 
      | for len=2:length(eventid_b)
      | Splitname=regexp(Event_Id,'_','all');
      | New_EventId=insertBefore(Event_Id,Splitname(end),num2str(len));
      | eval([char(New_EventId) '= 0;']);
      | set_param([eventid_b{len}],'Value',char(New_EventId));
      | end
      | 
      | %Set value of constant
      | set_param([dgnsw_b{:}],'Value',char(DiagROMFLAG));
      | % set_param([eventid_b{:}],'Value',[char(EventId) '_1']);
      | % set_param([eventid_b1{:}],'Value',[char(EventId) '_2']);
      | set_param([tsample_b{:}],'SampleTime',char(sample_time));
      | set_param([immt_b{:}],'Value',char(immediate));
      settings: AttributesFormatString=%<MaskType>\nEventId = %<EventId>\nDiagROMFLAG = %<DiagROMFLAG>\nsample_time = %<sample_time>\nimmediate = %<immediate>
      mask Help:
      | eval('path_lib=fileparts(which(''AEMS_Standard_Library''));');
      | doc_path = [path_lib '\help\AEMS_DEM_SET_EVENT_AVL_2D.pdf'];
      | eval('open(doc_path)')
      mask Display:
      | dgn_mask = ['Event ID: ' char(EventId) '\n Diagnosis ROMFLAG: ' char(DiagROMFLAG)];
      | 
      | disp(dgn_mask);
      | plot([5,5,5])
      | plot([6,6,6])
  AEMS_DEM_SET_EVENT_AVL_8D : Subsystem  Tag=[LIB]  mask(AEMS_DEM_SET_EVENT_AVL_8D){EventId=Dem_EventId_XXX, DiagROMFLAG=mfXXX, sample_time=-1}
      mask init:
      | %EventId is defined only in the library
      | % eval([char(EventId) '_1 = 0;'])
      | % eval([char(EventId) '_2 = 0;'])
      | % eval([char(EventId) '_3 = 0;'])
      | % eval([char(EventId) '_4 = 0;'])
      | % eval([char(EventId) '_5 = 0;'])
      | % eval([char(EventId) '_6 = 0;'])
      | % eval([char(EventId) '_7 = 0;'])
      | % eval([char(EventId) '_8 = 0;'])
      | 
      | %Specify constant block
      | dgnsw_b = find_system(gcb,'LookUnderMasks','all','FollowLinks','on','Name','Diagnosis_SW');
      | tsample_b = find_system(gcb,'LookUnderMasks','all','FollowLinks','on','Name','DEM_SET_EVENT_AVL_UD');
      | 
      | Event_Id=get_param(gcb,'EventId');
      | 
      | eventid_b = find_system(gcb,'LookUnderMasks','all','FollowLinks','on','regexp','on','Name','^EventId_block');
      | eventid_b1 = find_system(gcb,'LookUnderMasks','all','FollowLinks','on','Name','EventId_block1');
      | eval([char(Event_Id) '= 0;']);
      | set_param(eventid_b1{:},'Value',char(Event_Id));
      | 
      | for len=2:length(eventid_b)
      | Splitname=regexp(Event_Id,'_','all');
      | New_EventId=insertBefore(Event_Id,Splitname(end),num2str(len));
      | eval([char(New_EventId) '= 0;']);
      | set_param([eventid_b{len}],'Value',char(New_EventId));
      | end
      | 
      | %Set value of constant
      | set_param([dgnsw_b{:}],'Value',char(DiagROMFLAG));
      | set_param([tsample_b{:}],'SampleTime',char(sample_time));
      settings: AttributesFormatString=%<MaskType>\nEventId = %<EventId>\nDiagROMFLAG = %<DiagROMFLAG>\nsample_time = %<sample_time>
      mask Help:
      | eval('path_lib=fileparts(which(''AEMS_Standard_Library''));');
      | doc_path = [path_lib '\help\AEMS_DEM_SET_EVENT_AVL_8D.pdf'];
      | eval('open(doc_path)')
      mask Display:
      | dgn_mask = ['Event ID: ' char(EventId) '\n Diagnosis ROMFLAG: ' char(DiagROMFLAG)];
      | 
      | disp(dgn_mask);
      | plot([5,5,5])
      | plot([6,6,6])
  AEMS_DEM_SET_EVENT_AVL_9D : Subsystem  Tag=[LIB]  mask(AEMS_DEM_SET_EVENT_AVL_9D){EventId=Dem_EventId_XXX, DiagROMFLAG=mfXXX, sample_time=-1}
      mask init:
      | %EventId is defined only in the library
      | % eval([char(EventId) '_1 = 0;'])
      | % eval([char(EventId) '_2 = 0;'])
      | % eval([char(EventId) '_3 = 0;'])
      | % eval([char(EventId) '_4 = 0;'])
      | % eval([char(EventId) '_5 = 0;'])
      | % eval([char(EventId) '_6 = 0;'])
      | % eval([char(EventId) '_7 = 0;'])
      | % eval([char(EventId) '_8 = 0;'])
      | % eval([char(EventId) '_0 = 0;'])
      | 
      | %Specify constant block
      | dgnsw_b = find_system(gcb,'LookUnderMasks','all','FollowLinks','on','Name','Diagnosis_SW');
      | tsample_b = find_system(gcb,'LookUnderMasks','all','FollowLinks','on','Name','DEM_SET_EVENT_AVL_UD');
      | 
      | Event_Id=get_param(gcb,'EventId');
      | 
      | eventid_b = find_system(gcb,'LookUnderMasks','all','FollowLinks','on','regexp','on','Name','^EventId_block');
      | eventid_b0 = find_system(gcb,'LookUnderMasks','all','FollowLinks','on','Name','EventId_block0');
      | eval([char(Event_Id) '= 0;']);
      | set_param(eventid_b0{:},'Value',char(Event_Id));
      | 
      | for len=2:length(eventid_b)
      | Splitname=regexp(Event_Id,'_','all');
      | New_EventId=insertBefore(Event_Id,Splitname(end),num2str(len));
      | eval([char(New_EventId) '= 0;']);
      | set_param([eventid_b{len}],'Value',char(New_EventId));
      | end
      | 
      | 
      | %Set value of constant
      | set_param([dgnsw_b{:}],'Value',char(DiagROMFLAG));
      | set_param([tsample_b{:}],'SampleTime',char(sample_time));
      settings: AttributesFormatString=%<MaskType>\nEventId = %<EventId>\nDiagROMFLAG = %<DiagROMFLAG>\nsample_time = %<sample_time>
      mask Help:
      | eval('path_lib=fileparts(which(''AEMS_Standard_Library''));');
      | doc_path = [path_lib '\help\AEMS_DEM_SET_EVENT_AVL_9D.pdf'];
      | eval('open(doc_path)')
      mask Display:
      | dgn_mask = ['Event ID: ' char(EventId) '\n Diagnosis ROMFLAG: ' char(DiagROMFLAG)];
      | 
      | disp(dgn_mask);
      | plot([5,5,5])
      | plot([6,6,6])
  AEMS_DEM_SET_EVENT_DSBL_1D : Subsystem  Tag=[LIB]  mask(AEMS_DEM_SET_EVENT_DSBL_1D){EventId=Dem_EventId_XXX}
      mask prompts: EventId "EventId :"
      mask init:
      | eval([char(EventId) '= 0;'])
      | 
      | %Specify constant block
      | eventid_b = find_system(gcb,'LookUnderMasks','all','FollowLinks','on','Name','EventId_block');
      | %Set value of constant
      | set_param([eventid_b{:}],'Value',char(EventId));
      settings: AttributesFormatString=%<MaskType>\nEventId : = %<EventId>
      mask Display:
      | % dgn_mask = ['Diagnosis name: ' char(DiagName) '\n Event ID: ' char(EventId)];
      | dgn_mask = ['Event ID: ' char(EventId)];
      | 
      | disp(dgn_mask);
      | port_label('input',1,'set_flag');
      | plot([5,5,5])
      | plot([6,6,6])
  AEMS_DEM_SET_EVENT_DSBL_2D : Subsystem  Tag=[LIB]  mask(AEMS_DEM_SET_EVENT_DSBL_2D){EventId=Dem_EventId_XXX}
      mask prompts: EventId "EventId :"
      mask init:
      | % eval([char(EventId) '_1 = 0;'])
      | % eval([char(EventId) '_2 = 0;'])
      | lib_path = gcb;
      | 
      | Event_Id=get_param(lib_path,'EventId');
      | eventid_b = find_system(lib_path,'LookUnderMasks','all','FollowLinks','on','regexp','on','Name','^EventId_block');
      | eventid_b1 = find_system(lib_path,'LookUnderMasks','all','FollowLinks','on','Name','EventId_block1');
      | eval([char(Event_Id) ' = 0;']);
      | set_param([eventid_b1{:}],'Value',char(Event_Id));
      | 
      | Splitname=regexp(Event_Id,'_','all');
      | New_EventId=insertBefore(Event_Id,Splitname(end),num2str(2));
      | eval([char(New_EventId) ' = 0;']);
      | set_param([eventid_b{2}],'Value',char(New_EventId));
      settings: AttributesFormatString=%<MaskType>\nEventId : = %<EventId>
      mask Display:
      | % dgn_mask = ['Diagnosis name: ' char(DiagName) '\n Event ID: ' char(EventId)];
      | dgn_mask = ['Event ID: ' char(EventId)];
      | 
      | disp(dgn_mask);
      | port_label('input',1,'set_flag');
      | plot([5,5,5])
      | plot([6,6,6])
  AEMS_DEM_SET_EVENT_DSBL_8D : Subsystem  Tag=[LIB]  mask(AEMS_DEM_SET_EVENT_DSBL_8D){EventId=Dem_EventId_XXX}
      mask prompts: EventId "EventId :"
      mask init:
      | % eval([char(EventId) '_1 = 0;'])
      | % eval([char(EventId) '_2 = 0;'])
      | % eval([char(EventId) '_3 = 0;'])
      | % eval([char(EventId) '_4 = 0;'])
      | % eval([char(EventId) '_5 = 0;'])
      | % eval([char(EventId) '_6 = 0;'])
      | % eval([char(EventId) '_7 = 0;'])
      | % eval([char(EventId) '_8 = 0;'])
      | 
      | lib_path = gcb;
      | Event_Id=get_param(gcb,'EventId');
      | 
      | eventid_b = find_system(gcb,'LookUnderMasks','all','FollowLinks','on','regexp','on','Name','^EventId_block');
      | eventid_b1 = find_system(gcb,'LookUnderMasks','all','FollowLinks','on','Name','EventId_block1');
      | eval([char(Event_Id) ' = 0;']);
      | set_param(eventid_b1{:},'Value',char(Event_Id));
      | 
      | for len=2:length(eventid_b)
      | Splitname=regexp(Event_Id,'_','all');
      | New_EventId=insertBefore(Event_Id,Splitname(end),num2str(len));
      | eval([char(New_EventId) ' = 0;']);
      | set_param([eventid_b{len}],'Value',char(New_EventId));
      | end
      | 
      | % eventid_b1 = find_system(gcb,'LookUnderMasks','all','FollowLinks','on','Name','EventId_block1');
      | % eventid_b2 = find_system(gcb,'LookUnderMasks','all','FollowLinks','on','Name','EventId_block2');
      | % eventid_b3 = find_system(gcb,'LookUnderMasks','all','FollowLinks','on','Name','EventId_block3');
      | % eventid_b4 = find_system(gcb,'LookUnderMasks','all','FollowLinks','on','Name','EventId_block4');
      | % eventid_b5 = find_system(gcb,'LookUnderMasks','all','FollowLinks','on','Name','EventId_block5');
      | % eventid_b6 = find_system(gcb,'LookUnderMasks','all','FollowLinks','on','Name','EventId_block6');
      | % eventid_b7 = find_system(gcb,'LookUnderMasks','all','FollowLinks','on','Name','EventId_block7');
      | % eventid_b8 = find_system(gcb,'LookUnderMasks','all','FollowLinks','on','Name','EventId_block8');
      | % 
      | % set_param([eventid_b1{:}],'Value',[char(EventId) '_1']);
      | % set_param([eventid_b2{:}],'Value',[char(EventId) '_2']);
      | % set_param([eventid_b3{:}],'Value',[char(EventId) '_3']);
      | % set_param([eventid_b4{:}],'Value',[char(EventId) '_4']);
      | % set_param([eventid_b5{:}],'Value',[char(EventId) '_5']);
      | % set_param([eventid_b6{:}],'Value',[char(EventId) '_6']);
      | % set_param([eventid_b7{:}],'Value',[char(EventId) '_7']);
      | % set_param([eventid_b8{:}],'Value',[char(EventId) '_8']);
      settings: AttributesFormatString=%<MaskType>\nEventId : = %<EventId>
      mask Display:
      | % dgn_mask = ['Diagnosis name: ' char(DiagName) '\n Event ID: ' char(EventId)];
      | dgn_mask = ['Event ID: ' char(EventId)];
      | 
      | disp(dgn_mask);
      | port_label('input',1,'set_flag');
      | plot([5,5,5])
      | plot([6,6,6])
  AEMS_DEM_SET_EVENT_DSBL_9D : Subsystem  Tag=[LIB]  mask(AEMS_DEM_SET_EVENT_DSBL_9D){EventId=Dem_EventId_XXX}
      mask prompts: EventId "EventId :"
      mask init:
      | % eval([char(EventId) '_0 = 0;'])
      | % eval([char(EventId) '_1 = 0;'])
      | % eval([char(EventId) '_2 = 0;'])
      | % eval([char(EventId) '_3 = 0;'])
      | % eval([char(EventId) '_4 = 0;'])
      | % eval([char(EventId) '_5 = 0;'])
      | % eval([char(EventId) '_6 = 0;'])
      | % eval([char(EventId) '_7 = 0;'])
      | % eval([char(EventId) '_8 = 0;'])
      | 
      | lib_path = gcb;
      | Event_Id=get_param(gcb,'EventId');
      | 
      | eventid_b = find_system(gcb,'LookUnderMasks','all','FollowLinks','on','regexp','on','Name','^EventId_block');
      | eventid_b1 = find_system(gcb,'LookUnderMasks','all','FollowLinks','on','Name','EventId_block0');
      | eval([char(Event_Id) ' = 0;']);
      | set_param(eventid_b1{:},'Value',char(Event_Id));
      | 
      | for len=2:length(eventid_b)
      |     Splitname=regexp(Event_Id,'_','all');
      |     New_EventId=insertBefore(Event_Id,Splitname(end),num2str(len));
      |     eval([char(New_EventId) ' = 0;']);
      |     set_param([eventid_b{len}],'Value',char(New_EventId));
      | end
      | % eventid_b0 = find_system(gcb,'LookUnderMasks','all','FollowLinks','on','Name','EventId_block0');
      | % eventid_b1 = find_system(gcb,'LookUnderMasks','all','FollowLinks','on','Name','EventId_block1');
      | % eventid_b2 = find_system(gcb,'LookUnderMasks','all','FollowLinks','on','Name','EventId_block2');
      | % eventid_b3 = find_system(gcb,'LookUnderMasks','all','FollowLinks','on','Name','EventId_block3');
      | % eventid_b4 = find_system(gcb,'LookUnderMasks','all','FollowLinks','on','Name','EventId_block4');
      | % eventid_b5 = find_system(gcb,'LookUnderMasks','all','FollowLinks','on','Name','EventId_block5');
      | % eventid_b6 = find_system(gcb,'LookUnderMasks','all','FollowLinks','on','Name','EventId_block6');
      | % eventid_b7 = find_system(gcb,'LookUnderMasks','all','FollowLinks','on','Name','EventId_block7');
      | % eventid_b8 = find_system(gcb,'LookUnderMasks','all','FollowLinks','on','Name','EventId_block8');
      | % 
      | % set_param([eventid_b0{:}],'Value',[char(EventId) '_0']);
      | % set_param([eventid_b1{:}],'Value',[char(EventId) '_1']);
      | % set_param([eventid_b2{:}],'Value',[char(EventId) '_2']);
      | % set_param([eventid_b3{:}],'Value',[char(EventId) '_3']);
      | % set_param([eventid_b4{:}],'Value',[char(EventId) '_4']);
      | % set_param([eventid_b5{:}],'Value',[char(EventId) '_5']);
      | % set_param([eventid_b6{:}],'Value',[char(EventId) '_6']);
      | % set_param([eventid_b7{:}],'Value',[char(EventId) '_7']);
      | % set_param([eventid_b8{:}],'Value',[char(EventId) '_8']);
      settings: AttributesFormatString=%<MaskType>\nEventId : = %<EventId>
      mask Display:
      | dgn_mask = ['Event ID: ' char(EventId)];
      | 
      | disp(dgn_mask);
      | port_label('input',1,'set_flag');
      | plot([5,5,5])
      | plot([6,6,6])
  AEMS_DEM_SET_EVENT_STS_1D : Subsystem  Tag=[LIB]  mask(AEMS_DEM_SET_EVENT_STS_1D){EventId=Dem_EventId_XXX, LibType=_DGNTRP}
      mask prompts: EventId "EventId :"; LibType "DEM Library type :"
      mask init:
      | eval([char(EventId) '= 0;'])
      | 
      | eventid_b = find_system(gcb,'LookUnderMasks','all','FollowLinks','on','Name','EventId_block');
      | set_param([eventid_b{:}],'Value',char(EventId));
      | 
      | status_b = find_system(gcb,'LookUnderMasks','all','FollowLinks','on','Name','dgn_event_status_failed');
      | switch LibType
      |     case '_DGNTRP'
      |         set_param([status_b{:}],'Value','1');
      |     case '_DGNOK'
      |         set_param([status_b{:}],'Value','0');
      | end
      settings: AttributesFormatString=%<MaskType>\nEventId : = %<EventId>\nDEM Library type : = %<LibType>
      mask TypeOptions LibType: _DGNTRP | _DGNOK
      mask Display:
      | dgn_mask = ['Event ID: ' char(EventId) '\n Library type: ' char(LibType)];
      | 
      | disp(dgn_mask);
      | plot([5,5,5])
      | plot([6,6,6])
  AEMS_DEM_SET_EVENT_STS_2D : Subsystem  Tag=[LIB]  mask(AEMS_DEM_SET_EVENT_STS_2D){EventId=Dem_EventId_XXX, LibType=_DGNTRP}
      mask prompts: EventId "EventId :"; LibType "DEM Library type :"
      mask init:
      | % eval([char(EventId) '_1 = 0;'])
      | % eval([char(EventId) '_2 = 0;'])
      | 
      | Event_Id=get_param(gcb,'EventId');
      | 
      | eventid_b = find_system(gcb,'LookUnderMasks','all','FollowLinks','on','regexp','on','Name','^EventId_block');
      | eventid_b1 = find_system(gcb,'LookUnderMasks','all','FollowLinks','on','Name','EventId_block1');
      | eval([char(Event_Id) '= 0;']);
      | set_param(eventid_b1{:},'Value',char(Event_Id));
      | 
      | for len=2:length(eventid_b)
      |     Splitname=regexp(Event_Id,'_','all');
      |     New_EventId=insertBefore(Event_Id,Splitname(end),num2str(len));
      |     eval([char(New_EventId) '= 0;']);
      |     set_param([eventid_b{len}],'Value',char(New_EventId));
      | end
      | 
      | status_b1 = find_system(gcb,'LookUnderMasks','all','FollowLinks','on','Name','dgn_event_status_failed1');
      | status_b2 = find_system(gcb,'LookUnderMasks','all','FollowLinks','on','Name','dgn_event_status_failed2');
      | switch LibType
      |     case '_DGNTRP'
      |         set_param([status_b1{:}],'Value','1');
      |         set_param([status_b2{:}],'Value','1');
      |     case '_DGNOK'
      |         set_param([status_b1{:}],'Value','0');
      |         set_param([status_b2{:}],'Value','0');
      | end
      settings: AttributesFormatString=%<MaskType>\nEventId : = %<EventId>\nDEM Library type : = %<LibType>
      mask TypeOptions LibType: _DGNTRP | _DGNOK
      mask Display:
      | dgn_mask = ['Event ID: ' char(EventId) '\n Library type: ' char(LibType)];
      | 
      | disp(dgn_mask);
      | plot([5,5,5])
      | plot([6,6,6])
  AEMS_DEM_SET_EVENT_STS_8D : Subsystem  Tag=[LIB]  mask(AEMS_DEM_SET_EVENT_STS_8D){EventId=Dem_EventId_XXX, LibType=_DGNTRP}
      mask prompts: EventId "EventId :"; LibType "DEM Library type :"
      mask init:
      | Event_Id=get_param(gcb,'EventId');
      | 
      | eventid_b = find_system(gcb,'LookUnderMasks','all','FollowLinks','on','regexp','on','Name','^EventId_block');
      | eventid_b1 = find_system(gcb,'LookUnderMasks','all','FollowLinks','on','Name','EventId_block1');
      | eval([char(Event_Id) '= 0;']);
      | set_param(eventid_b1{:},'Value',char(Event_Id));
      | 
      | for len=2:length(eventid_b)
      | Splitname=regexp(Event_Id,'_','all');
      | New_EventId=insertBefore(Event_Id,Splitname(end),num2str(len));
      | eval([char(New_EventId) '= 0;']);
      | set_param([eventid_b{len}],'Value',char(New_EventId));
      | 
      | end
      | % eval([char(EventId) '_1 = 0;'])
      | % eval([char(EventId) '_2 = 0;'])
      | % eval([char(EventId) '_3 = 0;'])
      | % eval([char(EventId) '_4 = 0;'])
      | % eval([char(EventId) '_5 = 0;'])
      | % eval([char(EventId) '_6 = 0;'])
      | % eval([char(EventId) '_7 = 0;'])
      | % eval([char(EventId) '_8 = 0;'])
      | % 
      | % eventid_b1 = find_system(gcb,'LookUnderMasks','all','FollowLinks','on','Name','EventId_block1');
      | % eventid_b2 = find_system(gcb,'LookUnderMasks','all','FollowLinks','on','Name','EventId_block2');
      | % eventid_b3 = find_system(gcb,'LookUnderMasks','all','FollowLinks','on','Name','EventId_block3');
      | % eventid_b4 = find_system(gcb,'LookUnderMasks','all','FollowLinks','on','Name','EventId_block4');
      | % eventid_b5 = find_system(gcb,'LookUnderMasks','all','FollowLinks','on','Name','EventId_block5');
      | % eventid_b6 = find_system(gcb,'LookUnderMasks','all','FollowLinks','on','Name','EventId_block6');
      | % eventid_b7 = find_system(gcb,'LookUnderMasks','all','FollowLinks','on','Name','EventId_block7');
      | % eventid_b8 = find_system(gcb,'LookUnderMasks','all','FollowLinks','on','Name','EventId_block8');
      | % 
      | % set_param([eventid_b1{:}],'Value',[char(EventId) '_1']);
      | % set_param([eventid_b2{:}],'Value',[char(EventId) '_2']);
      | % set_param([eventid_b3{:}],'Value',[char(EventId) '_3']);
      | % set_param([eventid_b4{:}],'Value',[char(EventId) '_4']);
      | % set_param([eventid_b5{:}],'Value',[char(EventId) '_5']);
      | % set_param([eventid_b6{:}],'Value',[char(EventId) '_6']);
      | % set_param([eventid_b7{:}],'Value',[char(EventId) '_7']);
      | % set_param([eventid_b8{:}],'Value',[char(EventId) '_8']);
      | 
      | status_b1 = find_system(gcb,'LookUnderMasks','all','FollowLinks','on','Name','dgn_event_status_failed1');
      | status_b2 = find_system(gcb,'LookUnderMasks','all','FollowLinks','on','Name','dgn_event_status_failed2');
      | status_b3 = find_system(gcb,'LookUnderMasks','all','FollowLinks','on','Name','dgn_event_status_failed3');
      | status_b4 = find_system(gcb,'LookUnderMasks','all','FollowLinks','on','Name','dgn_event_status_failed4');
      | status_b5 = find_system(gcb,'LookUnderMasks','all','FollowLinks','on','Name','dgn_event_status_failed5');
      | status_b6 = find_system(gcb,'LookUnderMasks','all','FollowLinks','on','Name','dgn_event_status_failed6');
      | status_b7 = find_system(gcb,'LookUnderMasks','all','FollowLinks','on','Name','dgn_event_status_failed7');
      | status_b8 = find_system(gcb,'LookUnderMasks','all','FollowLinks','on','Name','dgn_event_status_failed8');
      | 
      | switch LibType
      |     case '_DGNTRP'
      |         set_param([status_b1{:}],'Value','1');
      |         set_param([status_b2{:}],'Value','1');
      |         set_param([status_b3{:}],'Value','1');
      |         set_param([status_b4{:}],'Value','1');
      |         set_param([status_b5{:}],'Value','1');
      |         set_param([status_b6{:}],'Value','1');
      |         set_param([status_b7{:}],'Value','1');
      |         set_param([status_b8{:}],'Value','1');
      |     case '_DGNOK'
      |         set_param([status_b1{:}],'Value','0');
      |         set_param([status_b2{:}],'Value','0');
      |         set_param([status_b3{:}],'Value','0');
      |         set_param([status_b4{:}],'Value','0');
      |         set_param([status_b5{:}],'Value','0');
      |         set_param([status_b6{:}],'Value','0');
      |         set_param([status_b7{:}],'Value','0');
      |         set_param([status_b8{:}],'Value','0');
      | end
      settings: AttributesFormatString=%<MaskType>\nEventId : = %<EventId>\nDEM Library type : = %<LibType>
      mask TypeOptions LibType: _DGNTRP | _DGNOK
      mask Display:
      | dgn_mask = ['Event ID: ' char(EventId) '\n Library type: ' char(LibType)];
      | 
      | disp(dgn_mask);
      | plot([5,5,5])
      | plot([6,6,6])
  AEMS_DEM_SET_EVENT_STS_9D : Subsystem  Tag=[LIB]  mask(AEMS_DEM_SET_EVENT_STS_9D){EventId=Dem_EventId_XXX, LibType=_DGNTRP}
      mask prompts: EventId "EventId :"; LibType "DEM Library type :"
      mask init:
      | Event_Id=get_param(gcb,'EventId');
      | 
      | eventid_b = find_system(gcb,'LookUnderMasks','all','FollowLinks','on','regexp','on','Name','^EventId_block');
      | eventid_b0 = find_system(gcb,'LookUnderMasks','all','FollowLinks','on','Name','EventId_block0');
      | eval([char(Event_Id) '= 0;']);
      | set_param(eventid_b0{:},'Value',char(Event_Id));
      | 
      | for len=2:length(eventid_b)
      |     Splitname=regexp(Event_Id,'_','all');
      |     New_EventId=insertBefore(Event_Id,Splitname(end),num2str(len));
      |     eval([char(New_EventId) '= 0;']);
      |     set_param([eventid_b{len}],'Value',char(New_EventId));
      | end
      | % eval([char(EventId) '_1 = 0;'])
      | % eval([char(EventId) '_2 = 0;'])
      | % eval([char(EventId) '_3 = 0;'])
      | % eval([char(EventId) '_4 = 0;'])
      | % eval([char(EventId) '_5 = 0;'])
      | % eval([char(EventId) '_6 = 0;'])
      | % eval([char(EventId) '_7 = 0;'])
      | % eval([char(EventId) '_8 = 0;'])
      | % eval([char(EventId) '_0 = 0;'])
      | % 
      | % eventid_b1 = find_system(gcb,'LookUnderMasks','all','FollowLinks','on','Name','EventId_block1');
      | % eventid_b2 = find_system(gcb,'LookUnderMasks','all','FollowLinks','on','Name','EventId_block2');
      | % eventid_b3 = find_system(gcb,'LookUnderMasks','all','FollowLinks','on','Name','EventId_block3');
      | % eventid_b4 = find_system(gcb,'LookUnderMasks','all','FollowLinks','on','Name','EventId_block4');
      | % eventid_b5 = find_system(gcb,'LookUnderMasks','all','FollowLinks','on','Name','EventId_block5');
      | % eventid_b6 = find_system(gcb,'LookUnderMasks','all','FollowLinks','on','Name','EventId_block6');
      | % eventid_b7 = find_system(gcb,'LookUnderMasks','all','FollowLinks','on','Name','EventId_block7');
      | % eventid_b8 = find_system(gcb,'LookUnderMasks','all','FollowLinks','on','Name','EventId_block8');
      | % eventid_b0 = find_system(gcb,'LookUnderMasks','all','FollowLinks','on','Name','EventId_block0');
      | % 
      | % set_param([eventid_b1{:}],'Value',[char(EventId) '_1']);
      | % set_param([eventid_b2{:}],'Value',[char(EventId) '_2']);
      | % set_param([eventid_b3{:}],'Value',[char(EventId) '_3']);
      | % set_param([eventid_b4{:}],'Value',[char(EventId) '_4']);
      | % set_param([eventid_b5{:}],'Value',[char(EventId) '_5']);
      | % set_param([eventid_b6{:}],'Value',[char(EventId) '_6']);
      | % set_param([eventid_b7{:}],'Value',[char(EventId) '_7']);
      | % set_param([eventid_b8{:}],'Value',[char(EventId) '_8']);
      | % set_param([eventid_b0{:}],'Value',[char(EventId) '_0']);
      | 
      | status_b1 = find_system(gcb,'LookUnderMasks','all','FollowLinks','on','Name','dgn_event_status_failed1');
      | status_b2 = find_system(gcb,'LookUnderMasks','all','FollowLinks','on','Name','dgn_event_status_failed2');
      | status_b3 = find_system(gcb,'LookUnderMasks','all','FollowLinks','on','Name','dgn_event_status_failed3');
      | status_b4 = find_system(gcb,'LookUnderMasks','all','FollowLinks','on','Name','dgn_event_status_failed4');
      | status_b5 = find_system(gcb,'LookUnderMasks','all','FollowLinks','on','Name','dgn_event_status_failed5');
      | status_b6 = find_system(gcb,'LookUnderMasks','all','FollowLinks','on','Name','dgn_event_status_failed6');
      | status_b7 = find_system(gcb,'LookUnderMasks','all','FollowLinks','on','Name','dgn_event_status_failed7');
      | status_b8 = find_system(gcb,'LookUnderMasks','all','FollowLinks','on','Name','dgn_event_status_failed8');
      | status_b0 = find_system(gcb,'LookUnderMasks','all','FollowLinks','on','Name','dgn_event_status_failed0');
      | 
      | switch LibType
      |     case '_DGNTRP'
      |         set_param([status_b1{:}],'Value','1');
      |         set_param([status_b2{:}],'Value','1');
      |         set_param([status_b3{:}],'Value','1');
      |         set_param([status_b4{:}],'Value','1');
      |         set_param([status_b5{:}],'Value','1');
      |         set_param([status_b6{:}],'Value','1');
      |         set_param([status_b7{:}],'Value','1');
      |         set_param([status_b8{:}],'Value','1');
      |         set_param([status_b0{:}],'Value','1');
      |     case '_DGNOK'
      |         set_param([status_b1{:}],'Value','0');
      |         set_param([status_b2{:}],'Value','0');
      |         set_param([status_b3{:}],'Value','0');
      |         set_param([status_b4{:}],'Value','0');
      |         set_param([status_b5{:}],'Value','0');
      |         set_param([status_b6{:}],'Value','0');
      |         set_param([status_b7{:}],'Value','0');
      |         set_param([status_b8{:}],'Value','0');
      |         set_param([status_b0{:}],'Value','0');
      | end
      settings: AttributesFormatString=%<MaskType>\nEventId : = %<EventId>\nDEM Library type : = %<LibType>
